simulink library "ammclib_bam"  (Simulink 9.3)
settings: Solver=VariableStepAuto  StartTime=0.0  StopTime=10.0  RelTol=1e-3
undefined symbols (not defined in the file): f16A1, f16A2, f16ADCMaxError, f16B0, f16B1, f16B2, f16C1, f16CC1, f16CC1sc, f16CC1sc_D, f16CC1sc_Q, f16CC2, f16CC2sc, f16CC2sc_D, f16CC2sc_Q, f16DerivGain, f16EGain, f16FiltCoef, f16HystOff, f16HystOn, f16IGain, f16IntegGain, f16IntegGainFW, f16IntegGainQ, f16Kd, f16Kq, f16Limit, f16LowerLimit, f16LowerLimit_D, f16LowerLimit_Q, f16LowerLimitFW, f16LowerLimitQ, f16ModIndex, f16OutValOff, f16OutValOn, f16PropGain, f16PropGainFW, f16PropGainQ, f16RampDown, f16RampUp, f16UGain, f16UpperLimit, f16UpperLimit_D, f16UpperLimit_Q, f16UpperLimitFW, f16UpperLimitQ, f16WIGain, f32A1, f32A2, f32ADCMaxError, f32B0, f32B1, f32B2, f32C1, f32CC1, f32CC1sc, f32CC1sc_D, f32CC1sc_Q, f32CC2, f32CC2sc ... (+62)
(part 2 of 15)

== system ammclib_bam/AMCLIB/F16 ==
  AMCLIB_BemfObsrvDQ_F16 : Subsystem  TreatAsAtomicUnit=on  mask(AMCLIB_BemfObsrvDQ_F16){showStates=Hide (faster execution), resetStatesEnable=Pre-set according to the first set of inputs after reset, f16IGain=0, f16UGain=0, f16WIGain=0, f16EGain=0, s16Shift=0, f16CC1sc_D=0, f16CC2sc_D=0, f16UpperLimit_D=0, f16LowerLimit_D=0, f16CC1sc_Q=0, f16CC2sc_Q=0, f16UpperLimit_Q=0, f16LowerLimit_Q=0, u16NShift=0}
      mask prompts: showStates "Show internal states"; resetStatesEnable "Internal state after reset"; f16IGain "f16IGain (Scaled RL circuit constant)"; f16UGain "f16UGain (Scaled voltage cross-coupling constant)"; f16WIGain "f16WIGain (Scaled angular velocity cross-coupling constant)"; f16EGain "f16EGain (Scaled back-EMF cross-coupling constant)"; s16Shift "s16Shift (Scaling bitwise shift applied to all cross-coupling constants)"; f16CC1sc_D "f16CC1sc_D (CC1 coefficient of the D-axis PI controller)"; f16CC2sc_D "f16CC2sc_D (CC2 coefficient of the D-axis PI controller)"; f16UpperLimit_D "f16UpperLimit_D (Upper Limit of the D-axis PI controller)"; f16LowerLimit_D "f16LowerLimit_D (Lower Limit of the D-axis PI controller)"; f16CC1sc_Q "f16CC1sc_Q (CC1 coefficient of the Q-axis PI controller)"; f16CC2sc_Q "f16CC2sc_Q (CC2 coefficient of the Q-axis PI controller)"; f16UpperLimit_Q "f16UpperLimit_Q (Upper Limit of the Q-axis PI controller)"; f16LowerLimit_Q "f16LowerLimit_Q (Lower Limit of the Q-axis PI controller)"; u16NShift "u16NShift (Scaling bitwise shift applied to the controller coefficients)"
      mask help: PMSM back-EMF observer DQ in 16-bit fixed-point fractional implementation. This block supports re-initialization of the internal state during simulation. If the block is reset, the observer will align with the motor's position and speed measured in the next time step. This allows seamless on-the-fly transition to the closed-loop control. Refer to the AMMCLIB User's Guide for further details.
      mask init:
      | if ~evalin('base','exist(''tS8'',''var'')')
      |   if (2 ~= exist('SWLIBS_Typedefs.mat','file'))
      |       error('File SWLIBS_Typedefs.mat is not on the Matlab path. Please add the AMMCLIB "bam" folder in the Matlab Search Path.');
      |   else
      |       evalin('base', 'load(''SWLIBS_Typedefs.mat'')');
      |   end
      | end
      | if showStates == 1
      |     % hidden state variables
      |     if strcmp(get_param([gcb '/f16IGain'], 'BlockType'), 'Inport')
      |         posblk = get_param(gcb, 'Position');
      | 
      |         pos = get_param(    [gcb, '/f16IGain'], 'Position');
      |         orient = get_param( [gcb, '/f16IGain'], 'Orientation');
      |         delete_block(       [gcb, '/f16IGain']);
      |         add_block('built-in/Ground', [gcb, '/f16IGain'], 'Position', pos, 'Orientation', orient);
      | 
      |         pos = get_param(    [gcb, '/f16UGain'], 'Position');
      |         orient = get_param( [gcb, '/f16UGain'], 'Orientation');
      |         delete_block(       [gcb, '/f16UGain']);
      |         add_block('built-in/Ground', [gcb, '/f16UGain'], 'Position', pos, 'Orientation', orient);
      | 
      |         pos = get_param(    [gcb, '/f16WIGain'], 'Position');
      |         orient = get_param( [gcb, '/f16WIGain'], 'Orientation');
      |         delete_block(       [gcb, '/f16WIGain']);
      |         add_block('built-in/Ground', [gcb, '/f16WIGain'], 'Position', pos, 'Orientation', orient);
      | 
      |         pos = get_param(    [gcb, '/f16EGain'], 'Position');
      |         orient = get_param( [gcb, '/f16EGain'], 'Orientation');
      |         delete_block(       [gcb, '/f16EGain']);
      |         add_block('built-in/Ground', [gcb, '/f16EGain'], 'Position', pos, 'Orientation', orient);
      | 
      |         pos = get_param(    [gcb, '/s16Shift'], 'Position');
      |         orient = get_param( [gcb, '/s16Shift'], 'Orientation');
      |         delete_block(       [gcb, '/s16Shift']);
      |         add_block('built-in/Ground', [gcb, '/s16Shift'], 'Position', pos, 'Orientation', orient);
      | 
      |         pos = get_param(    [gcb, '/f16CC1sc_D'], 'Position');
      |         orient = get_param( [gcb, '/f16CC1sc_D'], 'Orientation');
      |         delete_block(       [gcb, '/f16CC1sc_D']);
      |         add_block('built-in/Ground', [gcb, '/f16CC1sc_D'], 'Position', pos, 'Orientation', orient);
      | 
      |         pos = get_param(    [gcb, '/f16CC2sc_D'], 'Position');
      |         orient = get_param( [gcb, '/f16CC2sc_D'], 'Orientation');
      |         delete_block(       [gcb, '/f16CC2sc_D']);
      |         add_block('built-in/Ground', [gcb, '/f16CC2sc_D'], 'Position', pos, 'Orientation', orient);
      | 
      |         pos = get_param(    [gcb, '/f16UpperLimit_D'], 'Position');
      |         orient = get_param( [gcb, '/f16UpperLimit_D'], 'Orientation');
      |         delete_block(       [gcb, '/f16UpperLimit_D']);
      |         add_block('built-in/Ground', [gcb, '/f16UpperLimit_D'], 'Position', pos, 'Orientation', orient);
      | 
      |         pos = get_param(    [gcb, '/f16LowerLimit_D'], 'Position');
      |         orient = get_param( [gcb, '/f16LowerLimit_D'], 'Orientation');
      |         delete_block(       [gcb, '/f16LowerLimit_D']);
      |         add_block('built-in/Ground', [gcb, '/f16LowerLimit_D'], 'Position', pos, 'Orientation', orient);
      | 
      |         pos = get_param(    [gcb, '/f16CC1sc_Q'], 'Position');
      |         orient = get_param( [gcb, '/f16CC1sc_Q'], 'Orientation');
      |         delete_block(       [gcb, '/f16CC1sc_Q']);
      |         add_block('built-in/Ground', [gcb, '/f16CC1sc_Q'], 'Position', pos, 'Orientation', orient);
      | 
      |         pos = get_param(    [gcb, '/f16CC2sc_Q'], 'Position');
      |         orient = get_param( [gcb, '/f16CC2sc_Q'], 'Orientation');
      |         delete_block(       [gcb, '/f16CC2sc_Q']);
      |         add_block('built-in/Ground', [gcb, '/f16CC2sc_Q'], 'Position', pos, 'Orientation', orient);
      | 
      |         pos = get_param(    [gcb, '/f16UpperLimit_Q'], 'Position');
      |         orient = get_param( [gcb, '/f16UpperLimit_Q'], 'Orientation');
      |         delete_block(       [gcb, '/f16UpperLimit_Q']);
      |         add_block('built-in/Ground', [gcb, '/f16UpperLimit_Q'], 'Position', pos, 'Orientation', orient);
      | 
      |         pos = get_param(    [gcb, '/f16LowerLimit_Q'], 'Position');
      |         orient = get_param( [gcb, '/f16LowerLimit_Q'], 'Orientation');
      |         delete_block(       [gcb, '/f16LowerLimit_Q']);
      |         add_block('built-in/Ground', [gcb, '/f16LowerLimit_Q'], 'Position', pos, 'Orientation', orient);
      | 
      |         pos = get_param(    [gcb, '/u16NShift'], 'Position');
      |         orient = get_param( [gcb, '/u16NShift'], 'Orientation');
      |         delete_block(       [gcb, '/u16NShift']);
      |         add_block('built-in/Ground', [gcb, '/u16NShift'], 'Position', pos, 'Orientation', orient);
      | 
      |         pos = get_param(    [gcb, '/f32Acc_D'], 'Position');
      |         orient = get_param( [gcb, '/f32Acc_D'], 'Orientation');
      |         delete_block(       [gcb, '/f32Acc_D']);
      |         add_block('built-in/Ground', [gcb, '/f32Acc_D'], 'Position', pos, 'Orientation', orient);
      | 
      |         pos = get_param(    [gcb, '/f16InErrK1_D'], 'Position');
      |         orient = get_param( [gcb, '/f16InErrK1_D'], 'Orientation');
      |         delete_block(       [gcb, '/f16InErrK1_D']);
      |         add_block('built-in/Ground', [gcb, '/f16InErrK1_D'], 'Position', pos, 'Orientation', orient);
      | 
      |         pos = get_param(    [gcb, '/f32Acc_Q'], 'Position');
      |         orient = get_param( [gcb, '/f32Acc_Q'], 'Orientation');
      |         delete_block(       [gcb, '/f32Acc_Q']);
      |         add_block('built-in/Ground', [gcb, '/f32Acc_Q'], 'Position', pos, 'Orientation', orient);
      | 
      |         pos = get_param(    [gcb, '/f16InErrK1_Q'], 'Position');
      |         orient = get_param( [gcb, '/f16InErrK1_Q'], 'Orientation');
      |         delete_block(       [gcb, '/f16InErrK1_Q']);
      |         add_block('built-in/Ground', [gcb, '/f16InErrK1_Q'], 'Position', pos, 'Orientation', orient);
      | 
      |         pos = get_param(    [gcb, '/f32IObsrvIn_1L_D'], 'Position');
      |         orient = get_param( [gcb, '/f32IObsrvIn_1L_D'], 'Orientation');
      |         delete_block(       [gcb, '/f32IObsrvIn_1L_D']);
      |         add_block('built-in/Ground', [gcb, '/f32IObsrvIn_1L_D'], 'Position', pos, 'Orientation', orient);
      | 
      |         pos = get_param(    [gcb, '/f16IObsrvIn_1H_D'], 'Position');
      |         orient = get_param( [gcb, '/f16IObsrvIn_1H_D'], 'Orientation');
      |         delete_block(       [gcb, '/f16IObsrvIn_1H_D']);
      |         add_block('built-in/Ground', [gcb, '/f16IObsrvIn_1H_D'], 'Position', pos, 'Orientation', orient);
      | 
      |         pos = get_param(    [gcb, '/f32IObsrvIn_1L_Q'], 'Position');
      |         orient = get_param( [gcb, '/f32IObsrvIn_1L_Q'], 'Orientation');
      |         delete_block(       [gcb, '/f32IObsrvIn_1L_Q']);
      |         add_block('built-in/Ground', [gcb, '/f32IObsrvIn_1L_Q'], 'Position', pos, 'Orientation', orient);
      | 
      |         pos = get_param(    [gcb, '/f16IObsrvIn_1H_Q'], 'Position');
      |         orient = get_param( [gcb, '/f16IObsrvIn_1H_Q'], 'Orientation');
      |         delete_block(       [gcb, '/f16IObsrvIn_1H_Q']);
      |         add_block('built-in/Ground', [gcb, '/f16IObsrvIn_1H_Q'], 'Position', pos, 'Orientation', orient);
      | 
      |         pos = get_param(    [gcb, '/f32IObsrv_D'], 'Position');
      |         orient = get_param( [gcb, '/f32IObsrv_D'], 'Orientation');
      |         delete_block(       [gcb, '/f32IObsrv_D']);
      |         add_block('built-in/Ground', [gcb, '/f32IObsrv_D'], 'Position', pos, 'Orientation', orient);
      | 
      |         pos = get_param(    [gcb, '/f32IObsrv_Q'], 'Position');
      |         orient = get_param( [gcb, '/f32IObsrv_Q'], 'Orientation');
      |         delete_block(       [gcb, '/f32IObsrv_Q']);
      |         add_block('built-in/Ground', [gcb, '/f32IObsrv_Q'], 'Position', pos, 'Orientation', orient);
      | 
      | 
      |         pos = get_param(    [gcb '/f16EObsrv_D_Out'], 'Position');
      |         orient = get_param( [gcb '/f16EObsrv_D_Out'], 'Orientation');
      |         delete_block(       [gcb '/f16EObsrv_D_Out']);
      |         add_block('built-in/Terminator', [gcb '/f16EObsrv_D_Out'], 'Position', pos, 'Orientation', orient);
      | 
      |         pos = get_param(    [gcb '/f16EObsrv_Q_Out'], 'Position');
      |         orient = get_param( [gcb '/f16EObsrv_Q_Out'], 'Orientation');
      |         delete_block(       [gcb '/f16EObsrv_Q_Out']);
      |         add_block('built-in/Terminator', [gcb '/f16EObsrv_Q_Out'], 'Position', pos, 'Orientation', orient);
      | 
      |         pos = get_param(    [gcb '/f32Acc_D_Out'], 'Position');
      |         orient = get_param( [gcb '/f32Acc_D_Out'], 'Orientation');
      |         delete_block(       [gcb '/f32Acc_D_Out']);
      |         add_block('built-in/Terminator', [gcb '/f32Acc_D_Out'], 'Position', pos, 'Orientation', orient);
      | 
      |         pos = get_param(    [gcb '/f16InErrK1_D_Out'], 'Position');
      |         orient = get_param( [gcb '/f16InErrK1_D_Out'], 'Orientation');
      |         delete_block(       [gcb '/f16InErrK1_D_Out']);
      |         add_block('built-in/Terminator', [gcb '/f16InErrK1_D_Out'], 'Position', pos, 'Orientation', orient);
      | 
      |         pos = get_param(    [gcb '/f32Acc_Q_Out'], 'Position');
      |         orient = get_param( [gcb '/f32Acc_Q_Out'], 'Orientation');
      |         delete_block(       [gcb '/f32Acc_Q_Out']);
      |         add_block('built-in/Terminator', [gcb '/f32Acc_Q_Out'], 'Position', pos, 'Orientation', orient);
      | 
      |         pos = get_param(    [gcb '/f16InErrK1_Q_Out'], 'Position');
      |         orient = get_param( [gcb '/f16InErrK1_Q_Out'], 'Orientation');
      |         delete_block(       [gcb '/f16InErrK1_Q_Out']);
      |         add_block('built-in/Terminator', [gcb '/f16InErrK1_Q_Out'], 'Position', pos, 'Orientation', orient);
      | 
      |         pos = get_param(    [gcb '/f32IObsrvIn_1L_D_Out'], 'Position');
      |         orient = get_param( [gcb '/f32IObsrvIn_1L_D_Out'], 'Orientation');
      |         delete_block(       [gcb '/f32IObsrvIn_1L_D_Out']);
      |         add_block('built-in/Terminator', [gcb '/f32IObsrvIn_1L_D_Out'], 'Position', pos, 'Orientation', orient);
      | 
      |         pos = get_param(    [gcb '/f16IObsrvIn_1H_D_Out'], 'Position');
      |         orient = get_param( [gcb '/f16IObsrvIn_1H_D_Out'], 'Orientation');
      |         delete_block(       [gcb '/f16IObsrvIn_1H_D_Out']);
      |         add_block('built-in/Terminator', [gcb '/f16IObsrvIn_1H_D_Out'], 'Position', pos, 'Orientation', orient);
      | 
      |         pos = get_param(    [gcb '/f32IObsrvIn_1L_Q_Out'], 'Position');
      |         orient = get_param( [gcb '/f32IObsrvIn_1L_Q_Out'], 'Orientation');
      |         delete_block(       [gcb '/f32IObsrvIn_1L_Q_Out']);
      |         add_block('built-in/Terminator', [gcb '/f32IObsrvIn_1L_Q_Out'], 'Position', pos, 'Orientation', orient);
      | 
      |         pos = get_param(    [gcb '/f16IObsrvIn_1H_Q_Out'], 'Position');
      |         orient = get_param( [gcb '/f16IObsrvIn_1H_Q_Out'], 'Orientation');
      |         delete_block(       [gcb '/f16IObsrvIn_1H_Q_Out']);
      |         add_block('built-in/Terminator', [gcb '/f16IObsrvIn_1H_Q_Out'], 'Position', pos, 'Orientation', orient);
      | 
      |         pos = get_param(    [gcb '/f32IObsrv_D_Out'], 'Position');
      |         orient = get_param( [gcb '/f32IObsrv_D_Out'], 'Orientation');
      |         delete_block(       [gcb '/f32IObsrv_D_Out']);
      |         add_block('built-in/Terminator', [gcb '/f32IObsrv_D_Out'], 'Position', pos, 'Orientation', orient);
      | 
      |         pos = get_param(    [gcb '/f32IObsrv_Q_Out'], 'Position');
      |         orient = get_param( [gcb '/f32IObsrv_Q_Out'], 'Orientation');
      |         delete_block(       [gcb '/f32IObsrv_Q_Out']);
      |         add_block('built-in/Terminator', [gcb '/f32IObsrv_Q_Out'], 'Position', pos, 'Orientation', orient);
      | 
      | 
      |         set_param([gcb '/pIAB'], 'Port', '1');
      |         set_param([gcb '/pUAB'], 'Port', '2');
      |         set_param([gcb '/f16Velocity'], 'Port', '3');
      |         set_param([gcb '/f16Phase'], 'Port', '4');
      | 
      |         set_param([gcb '/f16PhaseErr'], 'Port', '1');
      | 
      |         set_param(gcb,'MaskEnables',{'on','on','on','on','on','on','on','on','on','on','on','on','on','on','on','on'});
      | 
      |         if (posblk(4) - posblk(2)) > 125
      |           height = 125;
      |           set_param(gcb,'Position',[posblk(1), posblk(2), posblk(3), posblk(2)+height])
      |         end
      |     end
      | else
      |     % shown state variables
      |     if strcmp(get_param([gcb '/f16IGain'], 'BlockType'), 'Ground')
      |         posblk = get_param(gcb, 'Position');
      | 
      |         pos = get_param(    [gcb, '/f16IGain'], 'Position');
      |         orient = get_param( [gcb, '/f16IGain'], 'Orientation');
      |         delete_block(       [gcb, '/f16IGain']);
      |         add_block('built-in/Inport', [gcb, '/f16IGain'], 'Position', pos, 'Orientation', orient, 'OutDataTypeStr', 'int16');
      | 
      |         pos = get_param(    [gcb, '/f16UGain'], 'Position');
      |         orient = get_param( [gcb, '/f16UGain'], 'Orientation');
      |         delete_block(       [gcb, '/f16UGain']);
      |         add_block('built-in/Inport', [gcb, '/f16UGain'], 'Position', pos, 'Orientation', orient, 'OutDataTypeStr', 'int16');
      | 
      |         pos = get_param(    [gcb, '/f16WIGain'], 'Position');
      |         orient = get_param( [gcb, '/f16WIGain'], 'Orientation');
      |         delete_block(       [gcb, '/f16WIGain']);
      |         add_block('built-in/Inport', [gcb, '/f16WIGain'], 'Position', pos, 'Orientation', orient, 'OutDataTypeStr', 'int16');
      | 
      |         pos = get_param(    [gcb, '/f16EGain'], 'Position');
      |         orient = get_param( [gcb, '/f16EGain'], 'Orientation');
      |         delete_block(       [gcb, '/f16EGain']);
      |         add_block('built-in/Inport', [gcb, '/f16EGain'], 'Position', pos, 'Orientation', orient, 'OutDataTypeStr', 'int16');
      | 
      |         pos = get_param(    [gcb, '/s16Shift'], 'Position');
      |         orient = get_param( [gcb, '/s16Shift'], 'Orientation');
      |         delete_block(       [gcb, '/s16Shift']);
      |         add_block('built-in/Inport', [gcb, '/s16Shift'], 'Position', pos, 'Orientation', orient, 'OutDataTypeStr', 'int16');
      | 
      |         pos = get_param(    [gcb, '/f16CC1sc_D'], 'Position');
      |         orient = get_param( [gcb, '/f16CC1sc_D'], 'Orientation');
      |         delete_block(       [gcb, '/f16CC1sc_D']);
      |         add_block('built-in/Inport', [gcb, '/f16CC1sc_D'], 'Position', pos, 'Orientation', orient, 'OutDataTypeStr', 'int16');
      | 
      |         pos = get_param(    [gcb, '/f16CC2sc_D'], 'Position');
      |         orient = get_param( [gcb, '/f16CC2sc_D'], 'Orientation');
      |         delete_block(       [gcb, '/f16CC2sc_D']);
      |         add_block('built-in/Inport', [gcb, '/f16CC2sc_D'], 'Position', pos, 'Orientation', orient, 'OutDataTypeStr', 'int16');
      | 
      |         pos = get_param(    [gcb, '/f16UpperLimit_D'], 'Position');
      |         orient = get_param( [gcb, '/f16UpperLimit_D'], 'Orientation');
      |         delete_block(       [gcb, '/f16UpperLimit_D']);
      |         add_block('built-in/Inport', [gcb, '/f16UpperLimit_D'], 'Position', pos, 'Orientation', orient, 'OutDataTypeStr', 'int16');
      | 
      |         pos = get_param(    [gcb, '/f16LowerLimit_D'], 'Position');
      |         orient = get_param( [gcb, '/f16LowerLimit_D'], 'Orientation');
      |         delete_block(       [gcb, '/f16LowerLimit_D']);
      |         add_block('built-in/Inport', [gcb, '/f16LowerLimit_D'], 'Position', pos, 'Orientation', orient, 'OutDataTypeStr', 'int16');
      | 
      |         pos = get_param(    [gcb, '/f16CC1sc_Q'], 'Position');
      |         orient = get_param( [gcb, '/f16CC1sc_Q'], 'Orientation');
      |         delete_block(       [gcb, '/f16CC1sc_Q']);
      |         add_block('built-in/Inport', [gcb, '/f16CC1sc_Q'], 'Position', pos, 'Orientation', orient, 'OutDataTypeStr', 'int16');
      | 
      |         pos = get_param(    [gcb, '/f16CC2sc_Q'], 'Position');
      |         orient = get_param( [gcb, '/f16CC2sc_Q'], 'Orientation');
      |         delete_block(       [gcb, '/f16CC2sc_Q']);
      |         add_block('built-in/Inport', [gcb, '/f16CC2sc_Q'], 'Position', pos, 'Orientation', orient, 'OutDataTypeStr', 'int16');
      | 
      |         pos = get_param(    [gcb, '/f16UpperLimit_Q'], 'Position');
      |         orient = get_param( [gcb, '/f16UpperLimit_Q'], 'Orientation');
      |         delete_block(       [gcb, '/f16UpperLimit_Q']);
      |         add_block('built-in/Inport', [gcb, '/f16UpperLimit_Q'], 'Position', pos, 'Orientation', orient, 'OutDataTypeStr', 'int16');
      | 
      |         pos = get_param(    [gcb, '/f16LowerLimit_Q'], 'Position');
      |         orient = get_param( [gcb, '/f16LowerLimit_Q'], 'Orientation');
      |         delete_block(       [gcb, '/f16LowerLimit_Q']);
      |         add_block('built-in/Inport', [gcb, '/f16LowerLimit_Q'], 'Position', pos, 'Orientation', orient, 'OutDataTypeStr', 'int16');
      | 
      |         pos = get_param(    [gcb, '/u16NShift'], 'Position');
      |         orient = get_param( [gcb, '/u16NShift'], 'Orientation');
      |         delete_block(       [gcb, '/u16NShift']);
      |         add_block('built-in/Inport', [gcb, '/u16NShift'], 'Position', pos, 'Orientation', orient, 'OutDataTypeStr', 'uint16');
      | 
      |         pos = get_param(    [gcb, '/f32Acc_D'], 'Position');
      |         orient = get_param( [gcb, '/f32Acc_D'], 'Orientation');
      |         delete_block(       [gcb, '/f32Acc_D']);
      |         add_block('built-in/Inport', [gcb, '/f32Acc_D'], 'Position', pos, 'Orientation', orient, 'OutDataTypeStr', 'int32');
      | 
      |         pos = get_param(    [gcb, '/f16InErrK1_D'], 'Position');
      |         orient = get_param( [gcb, '/f16InErrK1_D'], 'Orientation');
      |         delete_block(       [gcb, '/f16InErrK1_D']);
      |         add_block('built-in/Inport', [gcb, '/f16InErrK1_D'], 'Position', pos, 'Orientation', orient, 'OutDataTypeStr', 'int16');
      | 
      |         pos = get_param(    [gcb, '/f32Acc_Q'], 'Position');
      |         orient = get_param( [gcb, '/f32Acc_Q'], 'Orientation');
      |         delete_block(       [gcb, '/f32Acc_Q']);
      |         add_block('built-in/Inport', [gcb, '/f32Acc_Q'], 'Position', pos, 'Orientation', orient, 'OutDataTypeStr', 'int32');
      | 
      |         pos = get_param(    [gcb, '/f16InErrK1_Q'], 'Position');
      |         orient = get_param( [gcb, '/f16InErrK1_Q'], 'Orientation');
      |         delete_block(       [gcb, '/f16InErrK1_Q']);
      |         add_block('built-in/Inport', [gcb, '/f16InErrK1_Q'], 'Position', pos, 'Orientation', orient, 'OutDataTypeStr', 'int16');
      | 
      |         pos = get_param(    [gcb, '/f32IObsrvIn_1L_D'], 'Position');
      |         orient = get_param( [gcb, '/f32IObsrvIn_1L_D'], 'Orientation');
      |         delete_block(       [gcb, '/f32IObsrvIn_1L_D']);
      |         add_block('built-in/Inport', [gcb, '/f32IObsrvIn_1L_D'], 'Position', pos, 'Orientation', orient, 'OutDataTypeStr', 'int32');
      | 
      |         pos = get_param(    [gcb, '/f16IObsrvIn_1H_D'], 'Position');
      |         orient = get_param( [gcb, '/f16IObsrvIn_1H_D'], 'Orientation');
      |         delete_block(       [gcb, '/f16IObsrvIn_1H_D']);
      |         add_block('built-in/Inport', [gcb, '/f16IObsrvIn_1H_D'], 'Position', pos, 'Orientation', orient, 'OutDataTypeStr', 'int16');
      | 
      |         pos = get_param(    [gcb, '/f32IObsrvIn_1L_Q'], 'Position');
      |         orient = get_param( [gcb, '/f32IObsrvIn_1L_Q'], 'Orientation');
      |         delete_block(       [gcb, '/f32IObsrvIn_1L_Q']);
      |         add_block('built-in/Inport', [gcb, '/f32IObsrvIn_1L_Q'], 'Position', pos, 'Orientation', orient, 'OutDataTypeStr', 'int32');
      | 
      |         pos = get_param(    [gcb, '/f16IObsrvIn_1H_Q'], 'Position');
      |         orient = get_param( [gcb, '/f16IObsrvIn_1H_Q'], 'Orientation');
      |         delete_block(       [gcb, '/f16IObsrvIn_1H_Q']);
      |         add_block('built-in/Inport', [gcb, '/f16IObsrvIn_1H_Q'], 'Position', pos, 'Orientation', orient, 'OutDataTypeStr', 'int16');
      | 
      |         pos = get_param(    [gcb, '/f32IObsrv_D'], 'Position');
      |         orient = get_param( [gcb, '/f32IObsrv_D'], 'Orientation');
      |         delete_block(       [gcb, '/f32IObsrv_D']);
      |         add_block('built-in/Inport', [gcb, '/f32IObsrv_D'], 'Position', pos, 'Orientation', orient, 'OutDataTypeStr', 'int32');
      | 
      |         pos = get_param(    [gcb, '/f32IObsrv_Q'], 'Position');
      |         orient = get_param( [gcb, '/f32IObsrv_Q'], 'Orientation');
      |         delete_block(       [gcb, '/f32IObsrv_Q']);
      |         add_block('built-in/Inport', [gcb, '/f32IObsrv_Q'], 'Position', pos, 'Orientation', orient, 'OutDataTypeStr', 'int32');
      | 
      | 
      |         pos = get_param(    [gcb '/f16EObsrv_D_Out'], 'Position');
      |         orient = get_param( [gcb '/f16EObsrv_D_Out'], 'Orientation');
      |         delete_block(       [gcb '/f16EObsrv_D_Out']);
      |         add_block('built-in/Outport', [gcb '/f16EObsrv_D_Out'], 'Position', pos, 'Orientation', orient);
      | 
      |         pos = get_param(    [gcb '/f16EObsrv_Q_Out'], 'Position');
      |         orient = get_param( [gcb '/f16EObsrv_Q_Out'], 'Orientation');
      |         delete_block(       [gcb '/f16EObsrv_Q_Out']);
      |         add_block('built-in/Outport', [gcb '/f16EObsrv_Q_Out'], 'Position', pos, 'Orientation', orient);
      | 
      |         pos = get_param(    [gcb '/f32Acc_D_Out'], 'Position');
      |         orient = get_param( [gcb '/f32Acc_D_Out'], 'Orientation');
      |         delete_block(       [gcb '/f32Acc_D_Out']);
      |         add_block('built-in/Outport', [gcb '/f32Acc_D_Out'], 'Position', pos, 'Orientation', orient);
      | 
      |         pos = get_param(    [gcb '/f16InErrK1_D_Out'], 'Position');
      |         orient = get_param( [gcb '/f16InErrK1_D_Out'], 'Orientation');
      |         delete_block(       [gcb '/f16InErrK1_D_Out']);
      |         add_block('built-in/Outport', [gcb '/f16InErrK1_D_Out'], 'Position', pos, 'Orientation', orient);
      | 
      |         pos = get_param(    [gcb '/f32Acc_Q_Out'], 'Position');
      |         orient = get_param( [gcb '/f32Acc_Q_Out'], 'Orientation');
      |         delete_block(       [gcb '/f32Acc_Q_Out']);
      |         add_block('built-in/Outport', [gcb '/f32Acc_Q_Out'], 'Position', pos, 'Orientation', orient);
      | 
      |         pos = get_param(    [gcb '/f16InErrK1_Q_Out'], 'Position');
      |         orient = get_param( [gcb '/f16InErrK1_Q_Out'], 'Orientation');
      |         delete_block(       [gcb '/f16InErrK1_Q_Out']);
      |         add_block('built-in/Outport', [gcb '/f16InErrK1_Q_Out'], 'Position', pos, 'Orientation', orient);
      | 
      |         pos = get_param(    [gcb '/f32IObsrvIn_1L_D_Out'], 'Position');
      |         orient = get_param( [gcb '/f32IObsrvIn_1L_D_Out'], 'Orientation');
      |         delete_block(       [gcb '/f32IObsrvIn_1L_D_Out']);
      |         add_block('built-in/Outport', [gcb '/f32IObsrvIn_1L_D_Out'], 'Position', pos, 'Orientation', orient);
      | 
      |         pos = get_param(    [gcb '/f16IObsrvIn_1H_D_Out'], 'Position');
      |         orient = get_param( [gcb '/f16IObsrvIn_1H_D_Out'], 'Orientation');
      |         delete_block(       [gcb '/f16IObsrvIn_1H_D_Out']);
      |         add_block('built-in/Outport', [gcb '/f16IObsrvIn_1H_D_Out'], 'Position', pos, 'Orientation', orient);
      | 
      |         pos = get_param(    [gcb '/f32IObsrvIn_1L_Q_Out'], 'Position');
      |         orient = get_param( [gcb '/f32IObsrvIn_1L_Q_Out'], 'Orientation');
      |         delete_block(       [gcb '/f32IObsrvIn_1L_Q_Out']);
      |         add_block('built-in/Outport', [gcb '/f32IObsrvIn_1L_Q_Out'], 'Position', pos, 'Orientation', orient);
      | 
      |         pos = get_param(    [gcb '/f16IObsrvIn_1H_Q_Out'], 'Position');
      |         orient = get_param( [gcb '/f16IObsrvIn_1H_Q_Out'], 'Orientation');
      |         delete_block(       [gcb '/f16IObsrvIn_1H_Q_Out']);
      |         add_block('built-in/Outport', [gcb '/f16IObsrvIn_1H_Q_Out'], 'Position', pos, 'Orientation', orient);
      | 
      |         pos = get_param(    [gcb '/f32IObsrv_D_Out'], 'Position');
      |         orient = get_param( [gcb '/f32IObsrv_D_Out'], 'Orientation');
      |         delete_block(       [gcb '/f32IObsrv_D_Out']);
      |         add_block('built-in/Outport', [gcb '/f32IObsrv_D_Out'], 'Position', pos, 'Orientation', orient);
      | 
      |         pos = get_param(    [gcb '/f32IObsrv_Q_Out'], 'Position');
      |         orient = get_param( [gcb '/f32IObsrv_Q_Out'], 'Orientation');
      |         delete_block(       [gcb '/f32IObsrv_Q_Out']);
      |         add_block('built-in/Outport', [gcb '/f32IObsrv_Q_Out'], 'Position', pos, 'Orientation', orient);
      | 
      | 
      |         set_param([gcb '/pIAB'], 'Port', '1');
      |         set_param([gcb '/pUAB'], 'Port', '2');
      |         set_param([gcb '/f16Velocity'], 'Port', '3');
      |         set_param([gcb '/f16Phase'], 'Port', '4');
      |         set_param([gcb '/f16IGain'], 'Port', '5');
      |         set_param([gcb '/f16UGain'], 'Port', '6');
      |         set_param([gcb '/f16WIGain'], 'Port', '7');
      |         set_param([gcb '/f16EGain'], 'Port', '8');
      |         set_param([gcb '/s16Shift'], 'Port', '9');
      |         set_param([gcb '/f16CC1sc_D'], 'Port', '10');
      |         set_param([gcb '/f16CC2sc_D'], 'Port', '11');
      |         set_param([gcb '/f16UpperLimit_D'], 'Port', '12');
      |         set_param([gcb '/f16LowerLimit_D'], 'Port', '13');
      |         set_param([gcb '/f16CC1sc_Q'], 'Port', '14');
      |         set_param([gcb '/f16CC2sc_Q'], 'Port', '15');
      |         set_param([gcb '/f16UpperLimit_Q'], 'Port', '16');
      |         set_param([gcb '/f16LowerLimit_Q'], 'Port', '17');
      |         set_param([gcb '/u16NShift'], 'Port', '18');
      |         set_param([gcb '/f32Acc_D'], 'Port', '19');
      |         set_param([gcb '/f16InErrK1_D'], 'Port', '20');
      |         set_param([gcb '/f32Acc_Q'], 'Port', '21');
      |         set_param([gcb '/f16InErrK1_Q'], 'Port', '22');
      |         set_param([gcb '/f32IObsrvIn_1L_D'], 'Port', '23');
      |         set_param([gcb '/f16IObsrvIn_1H_D'], 'Port', '24');
      |         set_param([gcb '/f32IObsrvIn_1L_Q'], 'Port', '25');
      |         set_param([gcb '/f16IObsrvIn_1H_Q'], 'Port', '26');
      |         set_param([gcb '/f32IObsrv_D'], 'Port', '27');
      |         set_param([gcb '/f32IObsrv_Q'], 'Port', '28');
      | 
      |         set_param([gcb '/f16PhaseErr'], 'Port', '1');
      |         set_param([gcb '/f16EObsrv_D_Out'], 'Port', '2');
      |         set_param([gcb '/f16EObsrv_Q_Out'], 'Port', '3');
      |         set_param([gcb '/f32Acc_D_Out'], 'Port', '4');
      |         set_param([gcb '/f16InErrK1_D_Out'], 'Port', '5');
      |         set_param([gcb '/f32Acc_Q_Out'], 'Port', '6');
      |         set_param([gcb '/f16InErrK1_Q_Out'], 'Port', '7');
      |         set_param([gcb '/f32IObsrvIn_1L_D_Out'], 'Port', '8');
      |         set_param([gcb '/f16IObsrvIn_1H_D_Out'], 'Port', '9');
      |         set_param([gcb '/f32IObsrvIn_1L_Q_Out'], 'Port', '10');
      |         set_param([gcb '/f16IObsrvIn_1H_Q_Out'], 'Port', '11');
      |         set_param([gcb '/f32IObsrv_D_Out'], 'Port', '12');
      |         set_param([gcb '/f32IObsrv_Q_Out'], 'Port', '13');
      | 
      |         set_param(gcb,'MaskEnables',{'on','on','off','off','off','off','off','off','off','off','off','off','off','off','off','off'});
      | 
      |         if (posblk(4) - posblk(2)) < 725
      |           height = 725;
      |           set_param(gcb,'Position',[posblk(1), posblk(2), posblk(3), posblk(2)+height])
      |         end
      |     end
      | end
      settings: RTWSystemCode=Inline
      mask TypeOptions showStates: Hide (faster execution) | Show (allows debugging; connect feedback loops manually)
      mask Callback showStates:
      | maskStr = get_param(gcb,'showStates');
      | if strcmp(maskStr,'Hide (faster execution)'),
      |     set_param(gcb,'MaskEnables',{'on','on','on','on','on','on','on','on','on','on','on','on','on','on','on','on'});
      | else
      |     set_param(gcb,'MaskEnables',{'on','on','off','off','off','off','off','off','off','off','off','off','off','off','off','off'});
      | end
      mask TypeOptions resetStatesEnable: Pre-set according to the first set of inputs after reset | Clear to zero
      mask Display:
      | color('black');
      | pos = get_param(gcb, 'Position');
      | width = pos(3) - pos(1);
      | height = pos(4) - pos(2);
      | tX=width/2;
      | tY=height - 25;
      | color('black');
      | text(tX,tY, 'AMCLIB_BemfObsrvDQ_F16', 'horizontalAlignment', 'center');
      | if showStates == 2
      |   color('red');
      |   text(tX,tY - 20, ['debugging mode' char(13) char(10) '(limited performance)'], 'horizontalAlignment', 'center');
      | end
  AMCLIB_CurrentLoop_F16 : Subsystem  TreatAsAtomicUnit=on  mask(AMCLIB_CurrentLoop_F16){showStates=Hide (faster execution), resetStatesEnable=Pre-set according to the first set of inputs after reset, f16CC1sc_D=0, f16CC2sc_D=0, u16NShift_D=0, f16CC1sc_Q=0, f16CC2sc_Q=0, u16NShift_Q=0}
      mask prompts: showStates "Show internal states"; resetStatesEnable "Internal state after reset"; f16CC1sc_D "f16CC1sc_D (CC1 coefficient of the D-axis PI controller)"; f16CC2sc_D "f16CC2sc_D (CC2 coefficient of the D-axis PI controller)"; u16NShift_D "u16NShift_D (Scaling bitwise shift applied to the D-axis controller coefficients)"; f16CC1sc_Q "f16CC1sc_Q (CC1 coefficient of the Q-axis PI controller)"; f16CC2sc_Q "f16CC2sc_Q (CC2 coefficient of the Q-axis PI controller)"; u16NShift_Q "u16NShift_Q (Scaling bitwise shift applied to the Q-axis controller coefficients)"
      mask help: Current control loop of the PMSM field-oriented control algorithm in 16-bit fixed-point fractional implementation. This block supports re-initialization of the internal state during simulation. If the block is reset, the outputs of the PI controllers will be aligned with the inputs f16ControllerPIrAWDOut_preset and f16ControllerPIrAWQOut_preset. Refer to the AMMCLIB User's Guide for further details.
      mask init:
      | if ~evalin('base','exist(''tS8'',''var'')')
      |   if (2 ~= exist('SWLIBS_Typedefs.mat','file'))
      |       error('File SWLIBS_Typedefs.mat is not on the Matlab path. Please add the AMMCLIB "bam" folder in the Matlab Search Path.');
      |   else
      |       evalin('base', 'load(''SWLIBS_Typedefs.mat'')');
      |   end
      | end
      | if showStates == 1
      |     % hidden state variables
      |     if strcmp(get_param([gcb '/f16CC1sc_D'], 'BlockType'), 'Inport')
      |         posblk = get_param(gcb, 'Position');
      | 
      |         pos = get_param(    [gcb, '/f16CC1sc_D'], 'Position');
      |         orient = get_param( [gcb, '/f16CC1sc_D'], 'Orientation');
      |         delete_block(       [gcb, '/f16CC1sc_D']);
      |         add_block('built-in/Ground', [gcb, '/f16CC1sc_D'], 'Position', pos, 'Orientation', orient);
      | 
      |         pos = get_param(    [gcb, '/f16CC2sc_D'], 'Position');
      |         orient = get_param( [gcb, '/f16CC2sc_D'], 'Orientation');
      |         delete_block(       [gcb, '/f16CC2sc_D']);
      |         add_block('built-in/Ground', [gcb, '/f16CC2sc_D'], 'Position', pos, 'Orientation', orient);
      | 
      |         pos = get_param(    [gcb, '/u16NShift_D'], 'Position');
      |         orient = get_param( [gcb, '/u16NShift_D'], 'Orientation');
      |         delete_block(       [gcb, '/u16NShift_D']);
      |         add_block('built-in/Ground', [gcb, '/u16NShift_D'], 'Position', pos, 'Orientation', orient);
      | 
      |         pos = get_param(    [gcb, '/f16CC1sc_Q'], 'Position');
      |         orient = get_param( [gcb, '/f16CC1sc_Q'], 'Orientation');
      |         delete_block(       [gcb, '/f16CC1sc_Q']);
      |         add_block('built-in/Ground', [gcb, '/f16CC1sc_Q'], 'Position', pos, 'Orientation', orient);
      | 
      |         pos = get_param(    [gcb, '/f16CC2sc_Q'], 'Position');
      |         orient = get_param( [gcb, '/f16CC2sc_Q'], 'Orientation');
      |         delete_block(       [gcb, '/f16CC2sc_Q']);
      |         add_block('built-in/Ground', [gcb, '/f16CC2sc_Q'], 'Position', pos, 'Orientation', orient);
      | 
      |         pos = get_param(    [gcb, '/u16NShift_Q'], 'Position');
      |         orient = get_param( [gcb, '/u16NShift_Q'], 'Orientation');
      |         delete_block(       [gcb, '/u16NShift_Q']);
      |         add_block('built-in/Ground', [gcb, '/u16NShift_Q'], 'Position', pos, 'Orientation', orient);
      | 
      |         pos = get_param(    [gcb, '/f32Acc_D'], 'Position');
      |         orient = get_param( [gcb, '/f32Acc_D'], 'Orientation');
      |         delete_block(       [gcb, '/f32Acc_D']);
      |         add_block('built-in/Ground', [gcb, '/f32Acc_D'], 'Position', pos, 'Orientation', orient);
      | 
      |         pos = get_param(    [gcb, '/f16InErrK1_D'], 'Position');
      |         orient = get_param( [gcb, '/f16InErrK1_D'], 'Orientation');
      |         delete_block(       [gcb, '/f16InErrK1_D']);
      |         add_block('built-in/Ground', [gcb, '/f16InErrK1_D'], 'Position', pos, 'Orientation', orient);
      | 
      |         pos = get_param(    [gcb, '/f32Acc_Q'], 'Position');
      |         orient = get_param( [gcb, '/f32Acc_Q'], 'Orientation');
      |         delete_block(       [gcb, '/f32Acc_Q']);
      |         add_block('built-in/Ground', [gcb, '/f32Acc_Q'], 'Position', pos, 'Orientation', orient);
      | 
      |         pos = get_param(    [gcb, '/f16InErrK1_Q'], 'Position');
      |         orient = get_param( [gcb, '/f16InErrK1_Q'], 'Orientation');
      |         delete_block(       [gcb, '/f16InErrK1_Q']);
      |         add_block('built-in/Ground', [gcb, '/f16InErrK1_Q'], 'Position', pos, 'Orientation', orient);
      | 
      | 
      |         pos = get_param(    [gcb '/f32Acc_D_Out'], 'Position');
      |         orient = get_param( [gcb '/f32Acc_D_Out'], 'Orientation');
      |         delete_block(       [gcb '/f32Acc_D_Out']);
      |         add_block('built-in/Terminator', [gcb '/f32Acc_D_Out'], 'Position', pos, 'Orientation', orient);
      | 
      |         pos = get_param(    [gcb '/f16InErrK1_D_Out'], 'Position');
      |         orient = get_param( [gcb '/f16InErrK1_D_Out'], 'Orientation');
      |         delete_block(       [gcb '/f16InErrK1_D_Out']);
      |         add_block('built-in/Terminator', [gcb '/f16InErrK1_D_Out'], 'Position', pos, 'Orientation', orient);
      | 
      |         pos = get_param(    [gcb '/f32Acc_Q_Out'], 'Position');
      |         orient = get_param( [gcb '/f32Acc_Q_Out'], 'Orientation');
      |         delete_block(       [gcb '/f32Acc_Q_Out']);
      |         add_block('built-in/Terminator', [gcb '/f32Acc_Q_Out'], 'Position', pos, 'Orientation', orient);
      | 
      |         pos = get_param(    [gcb '/f16InErrK1_Q_Out'], 'Position');
      |         orient = get_param( [gcb '/f16InErrK1_Q_Out'], 'Orientation');
      |         delete_block(       [gcb '/f16InErrK1_Q_Out']);
      |         add_block('built-in/Terminator', [gcb '/f16InErrK1_Q_Out'], 'Position', pos, 'Orientation', orient);
      | 
      | 
      |         set_param([gcb '/f16UDcBus'], 'Port', '1');
      |         set_param([gcb '/pIDQReq'], 'Port', '2');
      |         set_param([gcb '/pIDQFbck'], 'Port', '3');
      |         set_param([gcb '/f16ControllerPIrAWDOut_preset'], 'Port', '4');
      |         set_param([gcb '/f16ControllerPIrAWQOut_preset'], 'Port', '5');
      | 
      |         set_param([gcb '/pUDQReq'], 'Port', '1');
      | 
      |         set_param(gcb,'MaskEnables',{'on','on','on','on','on','on','on','on'});
      | 
      |         if (posblk(4) - posblk(2)) > 150
      |           height = 150;
      |           set_param(gcb,'Position',[posblk(1), posblk(2), posblk(3), posblk(2)+height])
      |         end
      |     end
      | else
      |     % shown state variables
      |     if strcmp(get_param([gcb '/f16CC1sc_D'], 'BlockType'), 'Ground')
      |         posblk = get_param(gcb, 'Position');
      | 
      |         pos = get_param(    [gcb, '/f16CC1sc_D'], 'Position');
      |         orient = get_param( [gcb, '/f16CC1sc_D'], 'Orientation');
      |         delete_block(       [gcb, '/f16CC1sc_D']);
      |         add_block('built-in/Inport', [gcb, '/f16CC1sc_D'], 'Position', pos, 'Orientation', orient, 'OutDataTypeStr', 'int16');
      | 
      |         pos = get_param(    [gcb, '/f16CC2sc_D'], 'Position');
      |         orient = get_param( [gcb, '/f16CC2sc_D'], 'Orientation');
      |         delete_block(       [gcb, '/f16CC2sc_D']);
      |         add_block('built-in/Inport', [gcb, '/f16CC2sc_D'], 'Position', pos, 'Orientation', orient, 'OutDataTypeStr', 'int16');
      | 
      |         pos = get_param(    [gcb, '/u16NShift_D'], 'Position');
      |         orient = get_param( [gcb, '/u16NShift_D'], 'Orientation');
      |         delete_block(       [gcb, '/u16NShift_D']);
      |         add_block('built-in/Inport', [gcb, '/u16NShift_D'], 'Position', pos, 'Orientation', orient, 'OutDataTypeStr', 'uint16');
      | 
      |         pos = get_param(    [gcb, '/f16CC1sc_Q'], 'Position');
      |         orient = get_param( [gcb, '/f16CC1sc_Q'], 'Orientation');
      |         delete_block(       [gcb, '/f16CC1sc_Q']);
      |         add_block('built-in/Inport', [gcb, '/f16CC1sc_Q'], 'Position', pos, 'Orientation', orient, 'OutDataTypeStr', 'int16');
      | 
      |         pos = get_param(    [gcb, '/f16CC2sc_Q'], 'Position');
      |         orient = get_param( [gcb, '/f16CC2sc_Q'], 'Orientation');
      |         delete_block(       [gcb, '/f16CC2sc_Q']);
      |         add_block('built-in/Inport', [gcb, '/f16CC2sc_Q'], 'Position', pos, 'Orientation', orient, 'OutDataTypeStr', 'int16');
      | 
      |         pos = get_param(    [gcb, '/u16NShift_Q'], 'Position');
      |         orient = get_param( [gcb, '/u16NShift_Q'], 'Orientation');
      |         delete_block(       [gcb, '/u16NShift_Q']);
      |         add_block('built-in/Inport', [gcb, '/u16NShift_Q'], 'Position', pos, 'Orientation', orient, 'OutDataTypeStr', 'uint16');
      | 
      |         pos = get_param(    [gcb, '/f32Acc_D'], 'Position');
      |         orient = get_param( [gcb, '/f32Acc_D'], 'Orientation');
      |         delete_block(       [gcb, '/f32Acc_D']);
      |         add_block('built-in/Inport', [gcb, '/f32Acc_D'], 'Position', pos, 'Orientation', orient, 'OutDataTypeStr', 'int32');
      | 
      |         pos = get_param(    [gcb, '/f16InErrK1_D'], 'Position');
      |         orient = get_param( [gcb, '/f16InErrK1_D'], 'Orientation');
      |         delete_block(       [gcb, '/f16InErrK1_D']);
      |         add_block('built-in/Inport', [gcb, '/f16InErrK1_D'], 'Position', pos, 'Orientation', orient, 'OutDataTypeStr', 'int16');
      | 
      |         pos = get_param(    [gcb, '/f32Acc_Q'], 'Position');
      |         orient = get_param( [gcb, '/f32Acc_Q'], 'Orientation');
      |         delete_block(       [gcb, '/f32Acc_Q']);
      |         add_block('built-in/Inport', [gcb, '/f32Acc_Q'], 'Position', pos, 'Orientation', orient, 'OutDataTypeStr', 'int32');
      | 
      |         pos = get_param(    [gcb, '/f16InErrK1_Q'], 'Position');
      |         orient = get_param( [gcb, '/f16InErrK1_Q'], 'Orientation');
      |         delete_block(       [gcb, '/f16InErrK1_Q']);
      |         add_block('built-in/Inport', [gcb, '/f16InErrK1_Q'], 'Position', pos, 'Orientation', orient, 'OutDataTypeStr', 'int16');
      | 
      | 
      |         pos = get_param(    [gcb '/f32Acc_D_Out'], 'Position');
      |         orient = get_param( [gcb '/f32Acc_D_Out'], 'Orientation');
      |         delete_block(       [gcb '/f32Acc_D_Out']);
      |         add_block('built-in/Outport', [gcb '/f32Acc_D_Out'], 'Position', pos, 'Orientation', orient);
      | 
      |         pos = get_param(    [gcb '/f16InErrK1_D_Out'], 'Position');
      |         orient = get_param( [gcb '/f16InErrK1_D_Out'], 'Orientation');
      |         delete_block(       [gcb '/f16InErrK1_D_Out']);
      |         add_block('built-in/Outport', [gcb '/f16InErrK1_D_Out'], 'Position', pos, 'Orientation', orient);
      | 
      |         pos = get_param(    [gcb '/f32Acc_Q_Out'], 'Position');
      |         orient = get_param( [gcb '/f32Acc_Q_Out'], 'Orientation');
      |         delete_block(       [gcb '/f32Acc_Q_Out']);
      |         add_block('built-in/Outport', [gcb '/f32Acc_Q_Out'], 'Position', pos, 'Orientation', orient);
      | 
      |         pos = get_param(    [gcb '/f16InErrK1_Q_Out'], 'Position');
      |         orient = get_param( [gcb '/f16InErrK1_Q_Out'], 'Orientation');
      |         delete_block(       [gcb '/f16InErrK1_Q_Out']);
      |         add_block('built-in/Outport', [gcb '/f16InErrK1_Q_Out'], 'Position', pos, 'Orientation', orient);
      | 
      | 
      |         set_param([gcb '/f16UDcBus'], 'Port', '1');
      |         set_param([gcb '/pIDQReq'], 'Port', '2');
      |         set_param([gcb '/pIDQFbck'], 'Port', '3');
      |         set_param([gcb '/f16ControllerPIrAWDOut_preset'], 'Port', '4');
      |         set_param([gcb '/f16ControllerPIrAWQOut_preset'], 'Port', '5');
      |         set_param([gcb '/f16CC1sc_D'], 'Port', '6');
      |         set_param([gcb '/f16CC2sc_D'], 'Port', '7');
      |         set_param([gcb '/u16NShift_D'], 'Port', '8');
      |         set_param([gcb '/f16CC1sc_Q'], 'Port', '9');
      |         set_param([gcb '/f16CC2sc_Q'], 'Port', '10');
      |         set_param([gcb '/u16NShift_Q'], 'Port', '11');
      |         set_param([gcb '/f32Acc_D'], 'Port', '12');
      |         set_param([gcb '/f16InErrK1_D'], 'Port', '13');
      |         set_param([gcb '/f32Acc_Q'], 'Port', '14');
      |         set_param([gcb '/f16InErrK1_Q'], 'Port', '15');
      | 
      |         set_param([gcb '/pUDQReq'], 'Port', '1');
      |         set_param([gcb '/f32Acc_D_Out'], 'Port', '2');
      |         set_param([gcb '/f16InErrK1_D_Out'], 'Port', '3');
      |         set_param([gcb '/f32Acc_Q_Out'], 'Port', '4');
      |         set_param([gcb '/f16InErrK1_Q_Out'], 'Port', '5');
      | 
      |         set_param(gcb,'MaskEnables',{'on','on','off','off','off','off','off','off'});
      | 
      |         if (posblk(4) - posblk(2)) < 400
      |           height = 400;
      |           set_param(gcb,'Position',[posblk(1), posblk(2), posblk(3), posblk(2)+height])
      |         end
      |     end
      | end
      settings: RTWSystemCode=Inline
      mask TypeOptions showStates: Hide (faster execution) | Show (allows debugging; connect feedback loops manually)
      mask Callback showStates:
      | maskStr = get_param(gcb,'showStates');
      | if strcmp(maskStr,'Hide (faster execution)'),
      |     set_param(gcb,'MaskEnables',{'on','on','on','on','on','on','on','on'});
      | else
      |     set_param(gcb,'MaskEnables',{'on','on','off','off','off','off','off','off'});
      | end
      mask TypeOptions resetStatesEnable: Pre-set according to the first set of inputs after reset | Clear to zero
      mask Display:
      | color('black');
      | pos = get_param(gcb, 'Position');
      | width = pos(3) - pos(1);
      | height = pos(4) - pos(2);
      | tX=width/2;
      | tY=height - 25;
      | color('black');
      | text(tX,tY, 'AMCLIB_CurrentLoop_F16', 'horizontalAlignment', 'center');
      | if showStates == 2
      |   color('red');
      |   text(tX,tY - 20, ['debugging mode' char(13) char(10) '(limited performance)'], 'horizontalAlignment', 'center');
      | end
  AMCLIB_FWSpeedLoop_F16 : Subsystem  TreatAsAtomicUnit=on  mask(AMCLIB_FWSpeedLoop_F16){showStates=Hide (faster execution), resetStatesEnable=Pre-set according to the first set of inputs after reset, showDebugOutputs=Hide, u16NSamplesW=0, u16NSamplesFW=0, f16PropGainQ=0, f16IntegGainQ=0, s16PropGainShiftQ=0, s16IntegGainShiftQ=0, f16LowerLimitQ=0, f16UpperLimitQ=0, f16PropGainFW=0, f16IntegGainFW=0, s16PropGainShiftFW=0, s16IntegGainShiftFW=0, f16LowerLimitFW=0, f16UpperLimitFW=0, f32RampUp=0, f32RampDown=0}
      mask prompts: showStates "Show internal states"; resetStatesEnable "Internal state after reset"; showDebugOutputs "Show debugging outputs"; u16NSamplesW "u16NSamplesW (velocity GDFLIB_FilterMA - recalculated smoothing factor)"; u16NSamplesFW "u16NSamplesFW (FW GDFLIB_FilterMA - recalculated smoothing factor)"; f16PropGainQ "f16PropGainQ (q-axis GFLIB_ControllerPIpAW - proportional gain)"; f16IntegGainQ "f16IntegGainQ (q-axis GFLIB_ControllerPIpAW - integral gain)"; s16PropGainShiftQ "s16PropGainShiftQ (q-axis GFLIB_ControllerPIpAW - scaling bitwise shift applied to the proportional gain)"; s16IntegGainShiftQ "s16IntegGainShiftQ (q-axis GFLIB_ControllerPIpAW - scaling bitwise shift applied to the integral gain)"; f16LowerLimitQ "f16LowerLimitQ (q-axis GFLIB_ControllerPIpAW - lower limit)"; f16UpperLimitQ "f16UpperLimitQ (q-axis GFLIB_ControllerPIpAW - upper limit)"; f16PropGainFW "f16PropGainFW (FW GFLIB_ControllerPIpAW - proportional gain)"; f16IntegGainFW "f16IntegGainFW (FW GFLIB_ControllerPIpAW - integral gain)"; s16PropGainShiftFW "s16PropGainShiftFW (FW GFLIB_ControllerPIpAW - scaling bitwise shift applied to the proportional gain)"; s16IntegGainShiftFW "s16IntegGainShiftFW (FW GFLIB_ControllerPIpAW - scaling bitwise shift applied to the integral gain)"; f16LowerLimitFW "f16LowerLimitFW (FW GFLIB_ControllerPIpAW - lower limit)"; f16UpperLimitFW "f16UpperLimitFW (FW GFLIB_ControllerPIpAW - upper limit)"; f32RampUp "f32RampUp (Ramp up increment coefficient)"; f32RampDown "f32RampDown (Ramp decrement coefficient)"
      mask help: Speed loop controller with Field Weakening capability for the PMSM field-oriented control algorithm in 16-bit fixed-point fractional implementation. This block supports re-initialization of the internal state during simulation. If the block is reset, the outputs of the MA filters, PI controllers, and the ramp will be aligned with the inputs f16FilterMAWOut_preset, f16FilterMAFWOut_preset, f16ControllerPIpAWQOut_preset, f16ControllerPIpAWFWOut_preset, and f32RampOut_preset. Refer to the AMMCLIB User's Guide for further details.
      mask init:
      | if ~evalin('base','exist(''tS8'',''var'')')
      |   if (2 ~= exist('SWLIBS_Typedefs.mat','file'))
      |       error('File SWLIBS_Typedefs.mat is not on the Matlab path. Please add the AMMCLIB "bam" folder in the Matlab Search Path.');
      |   else
      |       evalin('base', 'load(''SWLIBS_Typedefs.mat'')');
      |   end
      | end
      | if showStates == 1
      |     % hidden state variables
      |     if strcmp(get_param([gcb '/u16NSamplesW'], 'BlockType'), 'Inport')
      |         posblk = get_param(gcb, 'Position');
      | 
      |         pos = get_param(    [gcb, '/u16NSamplesW'], 'Position');
      |         orient = get_param( [gcb, '/u16NSamplesW'], 'Orientation');
      |         delete_block(       [gcb, '/u16NSamplesW']);
      |         add_block('built-in/Ground', [gcb, '/u16NSamplesW'], 'Position', pos, 'Orientation', orient);
      | 
      |         pos = get_param(    [gcb, '/u16NSamplesFW'], 'Position');
      |         orient = get_param( [gcb, '/u16NSamplesFW'], 'Orientation');
      |         delete_block(       [gcb, '/u16NSamplesFW']);
      |         add_block('built-in/Ground', [gcb, '/u16NSamplesFW'], 'Position', pos, 'Orientation', orient);
      | 
      |         pos = get_param(    [gcb, '/f16PropGainQ'], 'Position');
      |         orient = get_param( [gcb, '/f16PropGainQ'], 'Orientation');
      |         delete_block(       [gcb, '/f16PropGainQ']);
      |         add_block('built-in/Ground', [gcb, '/f16PropGainQ'], 'Position', pos, 'Orientation', orient);
      | 
      |         pos = get_param(    [gcb, '/f16IntegGainQ'], 'Position');
      |         orient = get_param( [gcb, '/f16IntegGainQ'], 'Orientation');
      |         delete_block(       [gcb, '/f16IntegGainQ']);
      |         add_block('built-in/Ground', [gcb, '/f16IntegGainQ'], 'Position', pos, 'Orientation', orient);
      | 
      |         pos = get_param(    [gcb, '/s16PropGainShiftQ'], 'Position');
      |         orient = get_param( [gcb, '/s16PropGainShiftQ'], 'Orientation');
      |         delete_block(       [gcb, '/s16PropGainShiftQ']);
      |         add_block('built-in/Ground', [gcb, '/s16PropGainShiftQ'], 'Position', pos, 'Orientation', orient);
      | 
      |         pos = get_param(    [gcb, '/s16IntegGainShiftQ'], 'Position');
      |         orient = get_param( [gcb, '/s16IntegGainShiftQ'], 'Orientation');
      |         delete_block(       [gcb, '/s16IntegGainShiftQ']);
      |         add_block('built-in/Ground', [gcb, '/s16IntegGainShiftQ'], 'Position', pos, 'Orientation', orient);
      | 
      |         pos = get_param(    [gcb, '/f16LowerLimitQ'], 'Position');
      |         orient = get_param( [gcb, '/f16LowerLimitQ'], 'Orientation');
      |         delete_block(       [gcb, '/f16LowerLimitQ']);
      |         add_block('built-in/Ground', [gcb, '/f16LowerLimitQ'], 'Position', pos, 'Orientation', orient);
      | 
      |         pos = get_param(    [gcb, '/f16UpperLimitQ'], 'Position');
      |         orient = get_param( [gcb, '/f16UpperLimitQ'], 'Orientation');
      |         delete_block(       [gcb, '/f16UpperLimitQ']);
      |         add_block('built-in/Ground', [gcb, '/f16UpperLimitQ'], 'Position', pos, 'Orientation', orient);
      | 
      |         pos = get_param(    [gcb, '/f16PropGainFW'], 'Position');
      |         orient = get_param( [gcb, '/f16PropGainFW'], 'Orientation');
      |         delete_block(       [gcb, '/f16PropGainFW']);
      |         add_block('built-in/Ground', [gcb, '/f16PropGainFW'], 'Position', pos, 'Orientation', orient);
      | 
      |         pos = get_param(    [gcb, '/f16IntegGainFW'], 'Position');
      |         orient = get_param( [gcb, '/f16IntegGainFW'], 'Orientation');
      |         delete_block(       [gcb, '/f16IntegGainFW']);
      |         add_block('built-in/Ground', [gcb, '/f16IntegGainFW'], 'Position', pos, 'Orientation', orient);
      | 
      |         pos = get_param(    [gcb, '/s16PropGainShiftFW'], 'Position');
      |         orient = get_param( [gcb, '/s16PropGainShiftFW'], 'Orientation');
      |         delete_block(       [gcb, '/s16PropGainShiftFW']);
      |         add_block('built-in/Ground', [gcb, '/s16PropGainShiftFW'], 'Position', pos, 'Orientation', orient);
      | 
      |         pos = get_param(    [gcb, '/s16IntegGainShiftFW'], 'Position');
      |         orient = get_param( [gcb, '/s16IntegGainShiftFW'], 'Orientation');
      |         delete_block(       [gcb, '/s16IntegGainShiftFW']);
      |         add_block('built-in/Ground', [gcb, '/s16IntegGainShiftFW'], 'Position', pos, 'Orientation', orient);
      | 
      |         pos = get_param(    [gcb, '/f16LowerLimitFW'], 'Position');
      |         orient = get_param( [gcb, '/f16LowerLimitFW'], 'Orientation');
      |         delete_block(       [gcb, '/f16LowerLimitFW']);
      |         add_block('built-in/Ground', [gcb, '/f16LowerLimitFW'], 'Position', pos, 'Orientation', orient);
      | 
      |         pos = get_param(    [gcb, '/f16UpperLimitFW'], 'Position');
      |         orient = get_param( [gcb, '/f16UpperLimitFW'], 'Orientation');
      |         delete_block(       [gcb, '/f16UpperLimitFW']);
      |         add_block('built-in/Ground', [gcb, '/f16UpperLimitFW'], 'Position', pos, 'Orientation', orient);
      | 
      |         pos = get_param(    [gcb, '/f32RampUp'], 'Position');
      |         orient = get_param( [gcb, '/f32RampUp'], 'Orientation');
      |         delete_block(       [gcb, '/f32RampUp']);
      |         add_block('built-in/Ground', [gcb, '/f32RampUp'], 'Position', pos, 'Orientation', orient);
      | 
      |         pos = get_param(    [gcb, '/f32RampDown'], 'Position');
      |         orient = get_param( [gcb, '/f32RampDown'], 'Orientation');
      |         delete_block(       [gcb, '/f32RampDown']);
      |         add_block('built-in/Ground', [gcb, '/f32RampDown'], 'Position', pos, 'Orientation', orient);
      | 
      |         pos = get_param(    [gcb, '/f16IQReqK_1'], 'Position');
      |         orient = get_param( [gcb, '/f16IQReqK_1'], 'Orientation');
      |         delete_block(       [gcb, '/f16IQReqK_1']);
      |         add_block('built-in/Ground', [gcb, '/f16IQReqK_1'], 'Position', pos, 'Orientation', orient);
      | 
      |         pos = get_param(    [gcb, '/f32AccW'], 'Position');
      |         orient = get_param( [gcb, '/f32AccW'], 'Orientation');
      |         delete_block(       [gcb, '/f32AccW']);
      |         add_block('built-in/Ground', [gcb, '/f32AccW'], 'Position', pos, 'Orientation', orient);
      | 
      |         pos = get_param(    [gcb, '/f32AccFW'], 'Position');
      |         orient = get_param( [gcb, '/f32AccFW'], 'Orientation');
      |         delete_block(       [gcb, '/f32AccFW']);
      |         add_block('built-in/Ground', [gcb, '/f32AccFW'], 'Position', pos, 'Orientation', orient);
      | 
      |         pos = get_param(    [gcb, '/f32IntegPartK_1Q'], 'Position');
      |         orient = get_param( [gcb, '/f32IntegPartK_1Q'], 'Orientation');
      |         delete_block(       [gcb, '/f32IntegPartK_1Q']);
      |         add_block('built-in/Ground', [gcb, '/f32IntegPartK_1Q'], 'Position', pos, 'Orientation', orient);
      | 
      |         pos = get_param(    [gcb, '/f16InK_1Q'], 'Position');
      |         orient = get_param( [gcb, '/f16InK_1Q'], 'Orientation');
      |         delete_block(       [gcb, '/f16InK_1Q']);
      |         add_block('built-in/Ground', [gcb, '/f16InK_1Q'], 'Position', pos, 'Orientation', orient);
      | 
      |         pos = get_param(    [gcb, '/f32IntegPartK_1FW'], 'Position');
      |         orient = get_param( [gcb, '/f32IntegPartK_1FW'], 'Orientation');
      |         delete_block(       [gcb, '/f32IntegPartK_1FW']);
      |         add_block('built-in/Ground', [gcb, '/f32IntegPartK_1FW'], 'Position', pos, 'Orientation', orient);
      | 
      |         pos = get_param(    [gcb, '/f16InK_1FW'], 'Position');
      |         orient = get_param( [gcb, '/f16InK_1FW'], 'Orientation');
      |         delete_block(       [gcb, '/f16InK_1FW']);
      |         add_block('built-in/Ground', [gcb, '/f16InK_1FW'], 'Position', pos, 'Orientation', orient);
      | 
      |         pos = get_param(    [gcb, '/f32State'], 'Position');
      |         orient = get_param( [gcb, '/f32State'], 'Orientation');
      |         delete_block(       [gcb, '/f32State']);
      |         add_block('built-in/Ground', [gcb, '/f32State'], 'Position', pos, 'Orientation', orient);
      | 
      | 
      |         pos = get_param(    [gcb '/f32AccW_Out'], 'Position');
      |         orient = get_param( [gcb '/f32AccW_Out'], 'Orientation');
      |         delete_block(       [gcb '/f32AccW_Out']);
      |         add_block('built-in/Terminator', [gcb '/f32AccW_Out'], 'Position', pos, 'Orientation', orient);
      | 
      |         pos = get_param(    [gcb '/f32AccFW_Out'], 'Position');
      |         orient = get_param( [gcb '/f32AccFW_Out'], 'Orientation');
      |         delete_block(       [gcb '/f32AccFW_Out']);
      |         add_block('built-in/Terminator', [gcb '/f32AccFW_Out'], 'Position', pos, 'Orientation', orient);
      | 
      |         pos = get_param(    [gcb '/f32IntegPartK_1Q_Out'], 'Position');
      |         orient = get_param( [gcb '/f32IntegPartK_1Q_Out'], 'Orientation');
      |         delete_block(       [gcb '/f32IntegPartK_1Q_Out']);
      |         add_block('built-in/Terminator', [gcb '/f32IntegPartK_1Q_Out'], 'Position', pos, 'Orientation', orient);
      | 
      |         pos = get_param(    [gcb '/f16InK_1Q_Out'], 'Position');
      |         orient = get_param( [gcb '/f16InK_1Q_Out'], 'Orientation');
      |         delete_block(       [gcb '/f16InK_1Q_Out']);
      |         add_block('built-in/Terminator', [gcb '/f16InK_1Q_Out'], 'Position', pos, 'Orientation', orient);
      | 
      |         pos = get_param(    [gcb '/f32IntegPartK_1FW_Out'], 'Position');
      |         orient = get_param( [gcb '/f32IntegPartK_1FW_Out'], 'Orientation');
      |         delete_block(       [gcb '/f32IntegPartK_1FW_Out']);
      |         add_block('built-in/Terminator', [gcb '/f32IntegPartK_1FW_Out'], 'Position', pos, 'Orientation', orient);
      | 
      |         pos = get_param(    [gcb '/f16InK_1FW_Out'], 'Position');
      |         orient = get_param( [gcb '/f16InK_1FW_Out'], 'Orientation');
      |         delete_block(       [gcb '/f16InK_1FW_Out']);
      |         add_block('built-in/Terminator', [gcb '/f16InK_1FW_Out'], 'Position', pos, 'Orientation', orient);
      | 
      |         pos = get_param(    [gcb '/f32State_Out'], 'Position');
      |         orient = get_param( [gcb '/f32State_Out'], 'Orientation');
      |         delete_block(       [gcb '/f32State_Out']);
      |         add_block('built-in/Terminator', [gcb '/f32State_Out'], 'Position', pos, 'Orientation', orient);
      | 
      | 
      |         if strcmp(get_param([gcb '/f16WReqFilt'], 'BlockType'), 'Outport')
      |             pos = get_param(    [gcb '/f16WReqFilt'], 'Position');
      |             orient = get_param( [gcb '/f16WReqFilt'], 'Orientation');
      |             delete_block(       [gcb '/f16WReqFilt']);
      |             add_block('built-in/Terminator', [gcb '/f16WReqFilt'], 'Position', pos, 'Orientation', orient);
      | 
      |             pos = get_param(    [gcb '/f16WErr'], 'Position');
      |             orient = get_param( [gcb '/f16WErr'], 'Orientation');
      |             delete_block(       [gcb '/f16WErr']);
      |             add_block('built-in/Terminator', [gcb '/f16WErr'], 'Position', pos, 'Orientation', orient);
      | 
      |             pos = get_param(    [gcb '/f16IDQReqAmp'], 'Position');
      |             orient = get_param( [gcb '/f16IDQReqAmp'], 'Orientation');
      |             delete_block(       [gcb '/f16IDQReqAmp']);
      |             add_block('built-in/Terminator', [gcb '/f16IDQReqAmp'], 'Position', pos, 'Orientation', orient);
      | 
      |             pos = get_param(    [gcb '/f16WFbckFilt'], 'Position');
      |             orient = get_param( [gcb '/f16WFbckFilt'], 'Orientation');
      |             delete_block(       [gcb '/f16WFbckFilt']);
      |             add_block('built-in/Terminator', [gcb '/f16WFbckFilt'], 'Position', pos, 'Orientation', orient);
      | 
      |             pos = get_param(    [gcb '/f16IQErrSign'], 'Position');
      |             orient = get_param( [gcb '/f16IQErrSign'], 'Orientation');
      |             delete_block(       [gcb '/f16IQErrSign']);
      |             add_block('built-in/Terminator', [gcb '/f16IQErrSign'], 'Position', pos, 'Orientation', orient);
      | 
      |             pos = get_param(    [gcb '/f16IQErr'], 'Position');
      |             orient = get_param( [gcb '/f16IQErr'], 'Orientation');
      |             delete_block(       [gcb '/f16IQErr']);
      |             add_block('built-in/Terminator', [gcb '/f16IQErr'], 'Position', pos, 'Orientation', orient);
      | 
      |             pos = get_param(    [gcb '/f16FWErr'], 'Position');
      |             orient = get_param( [gcb '/f16FWErr'], 'Orientation');
      |             delete_block(       [gcb '/f16FWErr']);
      |             add_block('built-in/Terminator', [gcb '/f16FWErr'], 'Position', pos, 'Orientation', orient);
      | 
      |             pos = get_param(    [gcb '/f16UQErr'], 'Position');
      |             orient = get_param( [gcb '/f16UQErr'], 'Orientation');
      |             delete_block(       [gcb '/f16UQErr']);
      |             add_block('built-in/Terminator', [gcb '/f16UQErr'], 'Position', pos, 'Orientation', orient);
      | 
      |             pos = get_param(    [gcb '/f16FWErrFilt'], 'Position');
      |             orient = get_param( [gcb '/f16FWErrFilt'], 'Orientation');
      |             delete_block(       [gcb '/f16FWErrFilt']);
      |             add_block('built-in/Terminator', [gcb '/f16FWErrFilt'], 'Position', pos, 'Orientation', orient);
      | 
      |             pos = get_param(    [gcb '/f16FWAngle'], 'Position');
      |             orient = get_param( [gcb '/f16FWAngle'], 'Orientation');
      |             delete_block(       [gcb '/f16FWAngle']);
      |             add_block('built-in/Terminator', [gcb '/f16FWAngle'], 'Position', pos, 'Orientation', orient);
      | 
      |             pos = get_param(    [gcb '/f16FWSin'], 'Position');
      |             orient = get_param( [gcb '/f16FWSin'], 'Orientation');
      |             delete_block(       [gcb '/f16FWSin']);
      |             add_block('built-in/Terminator', [gcb '/f16FWSin'], 'Position', pos, 'Orientation', orient);
      | 
      |             pos = get_param(    [gcb '/f16FWCos'], 'Position');
      |             orient = get_param( [gcb '/f16FWCos'], 'Orientation');
      |             delete_block(       [gcb '/f16FWCos']);
      |             add_block('built-in/Terminator', [gcb '/f16FWCos'], 'Position', pos, 'Orientation', orient);
      | 
      |         end
      | 
      |         set_param([gcb '/f16VelocityReq'], 'Port', '1');
      |         set_param([gcb '/f16VelocityFbck'], 'Port', '2');
      |         set_param([gcb '/f16IQFbck'], 'Port', '3');
      |         set_param([gcb '/f16UQReq'], 'Port', '4');
      |         set_param([gcb '/f16UQLim'], 'Port', '5');
      |         set_param([gcb '/f16FilterMAWOut_preset'], 'Port', '6');
      |         set_param([gcb '/f16FilterMAFWOut_preset'], 'Port', '7');
      |         set_param([gcb '/f16ControllerPIpAWQOut_preset'], 'Port', '8');
      |         set_param([gcb '/f16ControllerPIpAWFWOut_preset'], 'Port', '9');
      |         set_param([gcb '/f32RampOut_preset'], 'Port', '10');
      | 
      |         set_param([gcb '/pIDQReq'], 'Port', '1');
      |         set_param([gcb '/u16LimitFlagQ'], 'Port', '2');
      |         set_param([gcb '/u16LimitFlagFW'], 'Port', '3');
      | 
      |         set_param(gcb,'MaskEnables',{'on','on','off','on','on','on','on','on','on','on','on','on','on','on','on','on','on','on','on'});
      | 
      |         if (posblk(4) - posblk(2)) > 275
      |           height = 275;
      |           set_param(gcb,'Position',[posblk(1), posblk(2), posblk(3), posblk(2)+height])
      |         end
      |     end
      | else
      |     % shown state variables
      |     if strcmp(get_param([gcb '/u16NSamplesW'], 'BlockType'), 'Ground')
      |         posblk = get_param(gcb, 'Position');
      | 
      |         pos = get_param(    [gcb, '/u16NSamplesW'], 'Position');
      |         orient = get_param( [gcb, '/u16NSamplesW'], 'Orientation');
      |         delete_block(       [gcb, '/u16NSamplesW']);
      |         add_block('built-in/Inport', [gcb, '/u16NSamplesW'], 'Position', pos, 'Orientation', orient, 'OutDataTypeStr', 'uint16');
      | 
      |         pos = get_param(    [gcb, '/u16NSamplesFW'], 'Position');
      |         orient = get_param( [gcb, '/u16NSamplesFW'], 'Orientation');
      |         delete_block(       [gcb, '/u16NSamplesFW']);
      |         add_block('built-in/Inport', [gcb, '/u16NSamplesFW'], 'Position', pos, 'Orientation', orient, 'OutDataTypeStr', 'uint16');
      | 
      |         pos = get_param(    [gcb, '/f16PropGainQ'], 'Position');
      |         orient = get_param( [gcb, '/f16PropGainQ'], 'Orientation');
      |         delete_block(       [gcb, '/f16PropGainQ']);
      |         add_block('built-in/Inport', [gcb, '/f16PropGainQ'], 'Position', pos, 'Orientation', orient, 'OutDataTypeStr', 'int16');
      | 
      |         pos = get_param(    [gcb, '/f16IntegGainQ'], 'Position');
      |         orient = get_param( [gcb, '/f16IntegGainQ'], 'Orientation');
      |         delete_block(       [gcb, '/f16IntegGainQ']);
      |         add_block('built-in/Inport', [gcb, '/f16IntegGainQ'], 'Position', pos, 'Orientation', orient, 'OutDataTypeStr', 'int16');
      | 
      |         pos = get_param(    [gcb, '/s16PropGainShiftQ'], 'Position');
      |         orient = get_param( [gcb, '/s16PropGainShiftQ'], 'Orientation');
      |         delete_block(       [gcb, '/s16PropGainShiftQ']);
      |         add_block('built-in/Inport', [gcb, '/s16PropGainShiftQ'], 'Position', pos, 'Orientation', orient, 'OutDataTypeStr', 'int16');
      | 
      |         pos = get_param(    [gcb, '/s16IntegGainShiftQ'], 'Position');
      |         orient = get_param( [gcb, '/s16IntegGainShiftQ'], 'Orientation');
      |         delete_block(       [gcb, '/s16IntegGainShiftQ']);
      |         add_block('built-in/Inport', [gcb, '/s16IntegGainShiftQ'], 'Position', pos, 'Orientation', orient, 'OutDataTypeStr', 'int16');
      | 
      |         pos = get_param(    [gcb, '/f16LowerLimitQ'], 'Position');
      |         orient = get_param( [gcb, '/f16LowerLimitQ'], 'Orientation');
      |         delete_block(       [gcb, '/f16LowerLimitQ']);
      |         add_block('built-in/Inport', [gcb, '/f16LowerLimitQ'], 'Position', pos, 'Orientation', orient, 'OutDataTypeStr', 'int16');
      | 
      |         pos = get_param(    [gcb, '/f16UpperLimitQ'], 'Position');
      |         orient = get_param( [gcb, '/f16UpperLimitQ'], 'Orientation');
      |         delete_block(       [gcb, '/f16UpperLimitQ']);
      |         add_block('built-in/Inport', [gcb, '/f16UpperLimitQ'], 'Position', pos, 'Orientation', orient, 'OutDataTypeStr', 'int16');
      | 
      |         pos = get_param(    [gcb, '/f16PropGainFW'], 'Position');
      |         orient = get_param( [gcb, '/f16PropGainFW'], 'Orientation');
      |         delete_block(       [gcb, '/f16PropGainFW']);
      |         add_block('built-in/Inport', [gcb, '/f16PropGainFW'], 'Position', pos, 'Orientation', orient, 'OutDataTypeStr', 'int16');
      | 
      |         pos = get_param(    [gcb, '/f16IntegGainFW'], 'Position');
      |         orient = get_param( [gcb, '/f16IntegGainFW'], 'Orientation');
      |         delete_block(       [gcb, '/f16IntegGainFW']);
      |         add_block('built-in/Inport', [gcb, '/f16IntegGainFW'], 'Position', pos, 'Orientation', orient, 'OutDataTypeStr', 'int16');
      | 
      |         pos = get_param(    [gcb, '/s16PropGainShiftFW'], 'Position');
      |         orient = get_param( [gcb, '/s16PropGainShiftFW'], 'Orientation');
      |         delete_block(       [gcb, '/s16PropGainShiftFW']);
      |         add_block('built-in/Inport', [gcb, '/s16PropGainShiftFW'], 'Position', pos, 'Orientation', orient, 'OutDataTypeStr', 'int16');
      | 
      |         pos = get_param(    [gcb, '/s16IntegGainShiftFW'], 'Position');
      |         orient = get_param( [gcb, '/s16IntegGainShiftFW'], 'Orientation');
      |         delete_block(       [gcb, '/s16IntegGainShiftFW']);
      |         add_block('built-in/Inport', [gcb, '/s16IntegGainShiftFW'], 'Position', pos, 'Orientation', orient, 'OutDataTypeStr', 'int16');
      | 
      |         pos = get_param(    [gcb, '/f16LowerLimitFW'], 'Position');
      |         orient = get_param( [gcb, '/f16LowerLimitFW'], 'Orientation');
      |         delete_block(       [gcb, '/f16LowerLimitFW']);
      |         add_block('built-in/Inport', [gcb, '/f16LowerLimitFW'], 'Position', pos, 'Orientation', orient, 'OutDataTypeStr', 'int16');
      | 
      |         pos = get_param(    [gcb, '/f16UpperLimitFW'], 'Position');
      |         orient = get_param( [gcb, '/f16UpperLimitFW'], 'Orientation');
      |         delete_block(       [gcb, '/f16UpperLimitFW']);
      |         add_block('built-in/Inport', [gcb, '/f16UpperLimitFW'], 'Position', pos, 'Orientation', orient, 'OutDataTypeStr', 'int16');
      | 
      |         pos = get_param(    [gcb, '/f32RampUp'], 'Position');
      |         orient = get_param( [gcb, '/f32RampUp'], 'Orientation');
      |         delete_block(       [gcb, '/f32RampUp']);
      |         add_block('built-in/Inport', [gcb, '/f32RampUp'], 'Position', pos, 'Orientation', orient, 'OutDataTypeStr', 'int32');
      | 
      |         pos = get_param(    [gcb, '/f32RampDown'], 'Position');
      |         orient = get_param( [gcb, '/f32RampDown'], 'Orientation');
      |         delete_block(       [gcb, '/f32RampDown']);
      |         add_block('built-in/Inport', [gcb, '/f32RampDown'], 'Position', pos, 'Orientation', orient, 'OutDataTypeStr', 'int32');
      | 
      |         pos = get_param(    [gcb, '/f16IQReqK_1'], 'Position');
      |         orient = get_param( [gcb, '/f16IQReqK_1'], 'Orientation');
      |         delete_block(       [gcb, '/f16IQReqK_1']);
      |         add_block('built-in/Inport', [gcb, '/f16IQReqK_1'], 'Position', pos, 'Orientation', orient, 'OutDataTypeStr', 'int16');
      | 
      |         pos = get_param(    [gcb, '/f32AccW'], 'Position');
      |         orient = get_param( [gcb, '/f32AccW'], 'Orientation');
      |         delete_block(       [gcb, '/f32AccW']);
      |         add_block('built-in/Inport', [gcb, '/f32AccW'], 'Position', pos, 'Orientation', orient, 'OutDataTypeStr', 'int32');
      | 
      |         pos = get_param(    [gcb, '/f32AccFW'], 'Position');
      |         orient = get_param( [gcb, '/f32AccFW'], 'Orientation');
      |         delete_block(       [gcb, '/f32AccFW']);
      |         add_block('built-in/Inport', [gcb, '/f32AccFW'], 'Position', pos, 'Orientation', orient, 'OutDataTypeStr', 'int32');
      | 
      |         pos = get_param(    [gcb, '/f32IntegPartK_1Q'], 'Position');
      |         orient = get_param( [gcb, '/f32IntegPartK_1Q'], 'Orientation');
      |         delete_block(       [gcb, '/f32IntegPartK_1Q']);
      |         add_block('built-in/Inport', [gcb, '/f32IntegPartK_1Q'], 'Position', pos, 'Orientation', orient, 'OutDataTypeStr', 'int32');
      | 
      |         pos = get_param(    [gcb, '/f16InK_1Q'], 'Position');
      |         orient = get_param( [gcb, '/f16InK_1Q'], 'Orientation');
      |         delete_block(       [gcb, '/f16InK_1Q']);
      |         add_block('built-in/Inport', [gcb, '/f16InK_1Q'], 'Position', pos, 'Orientation', orient, 'OutDataTypeStr', 'int16');
      | 
      |         pos = get_param(    [gcb, '/f32IntegPartK_1FW'], 'Position');
      |         orient = get_param( [gcb, '/f32IntegPartK_1FW'], 'Orientation');
      |         delete_block(       [gcb, '/f32IntegPartK_1FW']);
      |         add_block('built-in/Inport', [gcb, '/f32IntegPartK_1FW'], 'Position', pos, 'Orientation', orient, 'OutDataTypeStr', 'int32');
      | 
      |         pos = get_param(    [gcb, '/f16InK_1FW'], 'Position');
      |         orient = get_param( [gcb, '/f16InK_1FW'], 'Orientation');
      |         delete_block(       [gcb, '/f16InK_1FW']);
      |         add_block('built-in/Inport', [gcb, '/f16InK_1FW'], 'Position', pos, 'Orientation', orient, 'OutDataTypeStr', 'int16');
      | 
      |         pos = get_param(    [gcb, '/f32State'], 'Position');
      |         orient = get_param( [gcb, '/f32State'], 'Orientation');
      |         delete_block(       [gcb, '/f32State']);
      |         add_block('built-in/Inport', [gcb, '/f32State'], 'Position', pos, 'Orientation', orient, 'OutDataTypeStr', 'int32');
      | 
      | 
      |         pos = get_param(    [gcb '/f32AccW_Out'], 'Position');
      |         orient = get_param( [gcb '/f32AccW_Out'], 'Orientation');
      |         delete_block(       [gcb '/f32AccW_Out']);
      |         add_block('built-in/Outport', [gcb '/f32AccW_Out'], 'Position', pos, 'Orientation', orient);
      | 
      |         pos = get_param(    [gcb '/f32AccFW_Out'], 'Position');
      |         orient = get_param( [gcb '/f32AccFW_Out'], 'Orientation');
      |         delete_block(       [gcb '/f32AccFW_Out']);
      |         add_block('built-in/Outport', [gcb '/f32AccFW_Out'], 'Position', pos, 'Orientation', orient);
      | 
      |         pos = get_param(    [gcb '/f32IntegPartK_1Q_Out'], 'Position');
      |         orient = get_param( [gcb '/f32IntegPartK_1Q_Out'], 'Orientation');
      |         delete_block(       [gcb '/f32IntegPartK_1Q_Out']);
      |         add_block('built-in/Outport', [gcb '/f32IntegPartK_1Q_Out'], 'Position', pos, 'Orientation', orient);
      | 
      |         pos = get_param(    [gcb '/f16InK_1Q_Out'], 'Position');
      |         orient = get_param( [gcb '/f16InK_1Q_Out'], 'Orientation');
      |         delete_block(       [gcb '/f16InK_1Q_Out']);
      |         add_block('built-in/Outport', [gcb '/f16InK_1Q_Out'], 'Position', pos, 'Orientation', orient);
      | 
      |         pos = get_param(    [gcb '/f32IntegPartK_1FW_Out'], 'Position');
      |         orient = get_param( [gcb '/f32IntegPartK_1FW_Out'], 'Orientation');
      |         delete_block(       [gcb '/f32IntegPartK_1FW_Out']);
      |         add_block('built-in/Outport', [gcb '/f32IntegPartK_1FW_Out'], 'Position', pos, 'Orientation', orient);
      | 
      |         pos = get_param(    [gcb '/f16InK_1FW_Out'], 'Position');
      |         orient = get_param( [gcb '/f16InK_1FW_Out'], 'Orientation');
      |         delete_block(       [gcb '/f16InK_1FW_Out']);
      |         add_block('built-in/Outport', [gcb '/f16InK_1FW_Out'], 'Position', pos, 'Orientation', orient);
      | 
      |         pos = get_param(    [gcb '/f32State_Out'], 'Position');
      |         orient = get_param( [gcb '/f32State_Out'], 'Orientation');
      |         delete_block(       [gcb '/f32State_Out']);
      |         add_block('built-in/Outport', [gcb '/f32State_Out'], 'Position', pos, 'Orientation', orient);
      | 
      | 
      |         if (showDebugOutputs == 2) && (strcmp(get_param([gcb '/f16WReqFilt'], 'BlockType'), 'Terminator'))
      |             pos = get_param(    [gcb '/f16WReqFilt'], 'Position');
      |             orient = get_param( [gcb '/f16WReqFilt'], 'Orientation');
      |             delete_block(       [gcb '/f16WReqFilt']);
      |             add_block('built-in/Outport', [gcb '/f16WReqFilt'], 'Position', pos, 'Orientation', orient);
      | 
      |             pos = get_param(    [gcb '/f16WErr'], 'Position');
      |             orient = get_param( [gcb '/f16WErr'], 'Orientation');
      |             delete_block(       [gcb '/f16WErr']);
      |             add_block('built-in/Outport', [gcb '/f16WErr'], 'Position', pos, 'Orientation', orient);
      | 
      |             pos = get_param(    [gcb '/f16IDQReqAmp'], 'Position');
      |             orient = get_param( [gcb '/f16IDQReqAmp'], 'Orientation');
      |             delete_block(       [gcb '/f16IDQReqAmp']);
      |             add_block('built-in/Outport', [gcb '/f16IDQReqAmp'], 'Position', pos, 'Orientation', orient);
      | 
      |             pos = get_param(    [gcb '/f16WFbckFilt'], 'Position');
      |             orient = get_param( [gcb '/f16WFbckFilt'], 'Orientation');
      |             delete_block(       [gcb '/f16WFbckFilt']);
      |             add_block('built-in/Outport', [gcb '/f16WFbckFilt'], 'Position', pos, 'Orientation', orient);
      | 
      |             pos = get_param(    [gcb '/f16IQErrSign'], 'Position');
      |             orient = get_param( [gcb '/f16IQErrSign'], 'Orientation');
      |             delete_block(       [gcb '/f16IQErrSign']);
      |             add_block('built-in/Outport', [gcb '/f16IQErrSign'], 'Position', pos, 'Orientation', orient);
      | 
      |             pos = get_param(    [gcb '/f16IQErr'], 'Position');
      |             orient = get_param( [gcb '/f16IQErr'], 'Orientation');
      |             delete_block(       [gcb '/f16IQErr']);
      |             add_block('built-in/Outport', [gcb '/f16IQErr'], 'Position', pos, 'Orientation', orient);
      | 
      |             pos = get_param(    [gcb '/f16FWErr'], 'Position');
      |             orient = get_param( [gcb '/f16FWErr'], 'Orientation');
      |             delete_block(       [gcb '/f16FWErr']);
      |             add_block('built-in/Outport', [gcb '/f16FWErr'], 'Position', pos, 'Orientation', orient);
      | 
      |             pos = get_param(    [gcb '/f16UQErr'], 'Position');
      |             orient = get_param( [gcb '/f16UQErr'], 'Orientation');
      |             delete_block(       [gcb '/f16UQErr']);
      |             add_block('built-in/Outport', [gcb '/f16UQErr'], 'Position', pos, 'Orientation', orient);
      | 
      |             pos = get_param(    [gcb '/f16FWErrFilt'], 'Position');
      |             orient = get_param( [gcb '/f16FWErrFilt'], 'Orientation');
      |             delete_block(       [gcb '/f16FWErrFilt']);
      |             add_block('built-in/Outport', [gcb '/f16FWErrFilt'], 'Position', pos, 'Orientation', orient);
      | 
      |             pos = get_param(    [gcb '/f16FWAngle'], 'Position');
      |             orient = get_param( [gcb '/f16FWAngle'], 'Orientation');
      |             delete_block(       [gcb '/f16FWAngle']);
      |             add_block('built-in/Outport', [gcb '/f16FWAngle'], 'Position', pos, 'Orientation', orient);
      | 
      |             pos = get_param(    [gcb '/f16FWSin'], 'Position');
      |             orient = get_param( [gcb '/f16FWSin'], 'Orientation');
      |             delete_block(       [gcb '/f16FWSin']);
      |             add_block('built-in/Outport', [gcb '/f16FWSin'], 'Position', pos, 'Orientation', orient);
      | 
      |             pos = get_param(    [gcb '/f16FWCos'], 'Position');
      |             orient = get_param( [gcb '/f16FWCos'], 'Orientation');
      |             delete_block(       [gcb '/f16FWCos']);
      |             add_block('built-in/Outport', [gcb '/f16FWCos'], 'Position', pos, 'Orientation', orient);
      | 
      |         end
      | 
      |         set_param([gcb '/f16VelocityReq'], 'Port', '1');
      |         set_param([gcb '/f16VelocityFbck'], 'Port', '2');
      |         set_param([gcb '/f16IQFbck'], 'Port', '3');
      |         set_param([gcb '/f16UQReq'], 'Port', '4');
      |         set_param([gcb '/f16UQLim'], 'Port', '5');
      |         set_param([gcb '/f16FilterMAWOut_preset'], 'Port', '6');
      |         set_param([gcb '/f16FilterMAFWOut_preset'], 'Port', '7');
      |         set_param([gcb '/f16ControllerPIpAWQOut_preset'], 'Port', '8');
      |         set_param([gcb '/f16ControllerPIpAWFWOut_preset'], 'Port', '9');
      |         set_param([gcb '/f32RampOut_preset'], 'Port', '10');
      |         set_param([gcb '/u16NSamplesW'], 'Port', '11');
      |         set_param([gcb '/u16NSamplesFW'], 'Port', '12');
      |         set_param([gcb '/f16PropGainQ'], 'Port', '13');
      |         set_param([gcb '/f16IntegGainQ'], 'Port', '14');
      |         set_param([gcb '/s16PropGainShiftQ'], 'Port', '15');
      |         set_param([gcb '/s16IntegGainShiftQ'], 'Port', '16');
      |         set_param([gcb '/f16LowerLimitQ'], 'Port', '17');
      |         set_param([gcb '/f16UpperLimitQ'], 'Port', '18');
      |         set_param([gcb '/f16PropGainFW'], 'Port', '19');
      |         set_param([gcb '/f16IntegGainFW'], 'Port', '20');
      |         set_param([gcb '/s16PropGainShiftFW'], 'Port', '21');
      |         set_param([gcb '/s16IntegGainShiftFW'], 'Port', '22');
      |         set_param([gcb '/f16LowerLimitFW'], 'Port', '23');
      |         set_param([gcb '/f16UpperLimitFW'], 'Port', '24');
      |         set_param([gcb '/f32RampUp'], 'Port', '25');
      |         set_param([gcb '/f32RampDown'], 'Port', '26');
      |         set_param([gcb '/f16IQReqK_1'], 'Port', '27');
      |         set_param([gcb '/f32AccW'], 'Port', '28');
      |         set_param([gcb '/f32AccFW'], 'Port', '29');
      |         set_param([gcb '/f32IntegPartK_1Q'], 'Port', '30');
      |         set_param([gcb '/f16InK_1Q'], 'Port', '31');
      |         set_param([gcb '/f32IntegPartK_1FW'], 'Port', '32');
      |         set_param([gcb '/f16InK_1FW'], 'Port', '33');
      |         set_param([gcb '/f32State'], 'Port', '34');
      | 
      |         if (showDebugOutputs == 2)
      |             set_param([gcb '/pIDQReq'], 'Port', '1');
      |             set_param([gcb '/u16LimitFlagQ'], 'Port', '2');
      |             set_param([gcb '/u16LimitFlagFW'], 'Port', '3');
      |             set_param([gcb '/f16WReqFilt'], 'Port', '4');
      |             set_param([gcb '/f16WErr'], 'Port', '5');
      |             set_param([gcb '/f16IDQReqAmp'], 'Port', '6');
      |             set_param([gcb '/f16WFbckFilt'], 'Port', '7');
      |             set_param([gcb '/f16IQErrSign'], 'Port', '8');
      |             set_param([gcb '/f16IQErr'], 'Port', '9');
      |             set_param([gcb '/f16FWErr'], 'Port', '10');
      |             set_param([gcb '/f16UQErr'], 'Port', '11');
      |             set_param([gcb '/f16FWErrFilt'], 'Port', '12');
      |             set_param([gcb '/f16FWAngle'], 'Port', '13');
      |             set_param([gcb '/f16FWSin'], 'Port', '14');
      |             set_param([gcb '/f16FWCos'], 'Port', '15');
      |             set_param([gcb '/f32AccW_Out'], 'Port', '16');
      |             set_param([gcb '/f32AccFW_Out'], 'Port', '17');
      |             set_param([gcb '/f32IntegPartK_1Q_Out'], 'Port', '18');
      |             set_param([gcb '/f16InK_1Q_Out'], 'Port', '19');
      |             set_param([gcb '/f32IntegPartK_1FW_Out'], 'Port', '20');
      |             set_param([gcb '/f16InK_1FW_Out'], 'Port', '21');
      |             set_param([gcb '/f32State_Out'], 'Port', '22');
      |         else
      |             set_param([gcb '/pIDQReq'], 'Port', '1');
      |             set_param([gcb '/u16LimitFlagQ'], 'Port', '2');
      |             set_param([gcb '/u16LimitFlagFW'], 'Port', '3');
      |             set_param([gcb '/f32AccW_Out'], 'Port', '4');
      |             set_param([gcb '/f32AccFW_Out'], 'Port', '5');
      |             set_param([gcb '/f32IntegPartK_1Q_Out'], 'Port', '6');
      |             set_param([gcb '/f16InK_1Q_Out'], 'Port', '7');
      |             set_param([gcb '/f32IntegPartK_1FW_Out'], 'Port', '8');
      |             set_param([gcb '/f16InK_1FW_Out'], 'Port', '9');
      |             set_param([gcb '/f32State_Out'], 'Port', '10');
      |         end
      | 
      |         set_param(gcb,'MaskEnables',{'on','on','on','off','off','off','off','off','off','off','off','off','off','off','off','off','off','off','off'});
      | 
      |         if (posblk(4) - posblk(2)) < 875
      |           height = 875;
      |           set_param(gcb,'Position',[posblk(1), posblk(2), posblk(3), posblk(2)+height])
      |         end
      |     else
      |         if (showDebugOutputs == 2) && (strcmp(get_param([gcb '/f16WReqFilt'], 'BlockType'), 'Terminator'))
      |             % shown debugging outputs
      |             pos = get_param(    [gcb '/f16WReqFilt'], 'Position');
      |             orient = get_param( [gcb '/f16WReqFilt'], 'Orientation');
      |             delete_block(       [gcb '/f16WReqFilt']);
      |             add_block('built-in/Outport', [gcb '/f16WReqFilt'], 'Position', pos, 'Orientation', orient);
      | 
      |             pos = get_param(    [gcb '/f16WErr'], 'Position');
      |             orient = get_param( [gcb '/f16WErr'], 'Orientation');
      |             delete_block(       [gcb '/f16WErr']);
      |             add_block('built-in/Outport', [gcb '/f16WErr'], 'Position', pos, 'Orientation', orient);
      | 
      |             pos = get_param(    [gcb '/f16IDQReqAmp'], 'Position');
      |             orient = get_param( [gcb '/f16IDQReqAmp'], 'Orientation');
      |             delete_block(       [gcb '/f16IDQReqAmp']);
      |             add_block('built-in/Outport', [gcb '/f16IDQReqAmp'], 'Position', pos, 'Orientation', orient);
      | 
      |             pos = get_param(    [gcb '/f16WFbckFilt'], 'Position');
      |             orient = get_param( [gcb '/f16WFbckFilt'], 'Orientation');
      |             delete_block(       [gcb '/f16WFbckFilt']);
      |             add_block('built-in/Outport', [gcb '/f16WFbckFilt'], 'Position', pos, 'Orientation', orient);
      | 
      |             pos = get_param(    [gcb '/f16IQErrSign'], 'Position');
      |             orient = get_param( [gcb '/f16IQErrSign'], 'Orientation');
      |             delete_block(       [gcb '/f16IQErrSign']);
      |             add_block('built-in/Outport', [gcb '/f16IQErrSign'], 'Position', pos, 'Orientation', orient);
      | 
      |             pos = get_param(    [gcb '/f16IQErr'], 'Position');
      |             orient = get_param( [gcb '/f16IQErr'], 'Orientation');
      |             delete_block(       [gcb '/f16IQErr']);
      |             add_block('built-in/Outport', [gcb '/f16IQErr'], 'Position', pos, 'Orientation', orient);
      | 
      |             pos = get_param(    [gcb '/f16FWErr'], 'Position');
      |             orient = get_param( [gcb '/f16FWErr'], 'Orientation');
      |             delete_block(       [gcb '/f16FWErr']);
      |             add_block('built-in/Outport', [gcb '/f16FWErr'], 'Position', pos, 'Orientation', orient);
      | 
      |             pos = get_param(    [gcb '/f16UQErr'], 'Position');
      |             orient = get_param( [gcb '/f16UQErr'], 'Orientation');
      |             delete_block(       [gcb '/f16UQErr']);
      |             add_block('built-in/Outport', [gcb '/f16UQErr'], 'Position', pos, 'Orientation', orient);
      | 
      |             pos = get_param(    [gcb '/f16FWErrFilt'], 'Position');
      |             orient = get_param( [gcb '/f16FWErrFilt'], 'Orientation');
      |             delete_block(       [gcb '/f16FWErrFilt']);
      |             add_block('built-in/Outport', [gcb '/f16FWErrFilt'], 'Position', pos, 'Orientation', orient);
      | 
      |             pos = get_param(    [gcb '/f16FWAngle'], 'Position');
      |             orient = get_param( [gcb '/f16FWAngle'], 'Orientation');
      |             delete_block(       [gcb '/f16FWAngle']);
      |             add_block('built-in/Outport', [gcb '/f16FWAngle'], 'Position', pos, 'Orientation', orient);
      | 
      |             pos = get_param(    [gcb '/f16FWSin'], 'Position');
      |             orient = get_param( [gcb '/f16FWSin'], 'Orientation');
      |             delete_block(       [gcb '/f16FWSin']);
      |             add_block('built-in/Outport', [gcb '/f16FWSin'], 'Position', pos, 'Orientation', orient);
      | 
      |             pos = get_param(    [gcb '/f16FWCos'], 'Position');
      |             orient = get_param( [gcb '/f16FWCos'], 'Orientation');
      |             delete_block(       [gcb '/f16FWCos']);
      |             add_block('built-in/Outport', [gcb '/f16FWCos'], 'Position', pos, 'Orientation', orient);
      | 
      |             set_param([gcb '/pIDQReq'], 'Port', '1');
      |             set_param([gcb '/u16LimitFlagQ'], 'Port', '2');
      |             set_param([gcb '/u16LimitFlagFW'], 'Port', '3');
      |             set_param([gcb '/f16WReqFilt'], 'Port', '4');
      |             set_param([gcb '/f16WErr'], 'Port', '5');
      |             set_param([gcb '/f16IDQReqAmp'], 'Port', '6');
      |             set_param([gcb '/f16WFbckFilt'], 'Port', '7');
      |             set_param([gcb '/f16IQErrSign'], 'Port', '8');
      |             set_param([gcb '/f16IQErr'], 'Port', '9');
      |             set_param([gcb '/f16FWErr'], 'Port', '10');
      |             set_param([gcb '/f16UQErr'], 'Port', '11');
      |             set_param([gcb '/f16FWErrFilt'], 'Port', '12');
      |             set_param([gcb '/f16FWAngle'], 'Port', '13');
      |             set_param([gcb '/f16FWSin'], 'Port', '14');
      |             set_param([gcb '/f16FWCos'], 'Port', '15');
      |             set_param([gcb '/f32AccW_Out'], 'Port', '16');
      |             set_param([gcb '/f32AccFW_Out'], 'Port', '17');
      |             set_param([gcb '/f32IntegPartK_1Q_Out'], 'Port', '18');
      |             set_param([gcb '/f16InK_1Q_Out'], 'Port', '19');
      |             set_param([gcb '/f32IntegPartK_1FW_Out'], 'Port', '20');
      |             set_param([gcb '/f16InK_1FW_Out'], 'Port', '21');
      |             set_param([gcb '/f32State_Out'], 'Port', '22');
      |         elseif (showDebugOutputs == 1) && (strcmp(get_param([gcb '/f16WReqFilt'], 'BlockType'), 'Outport'))
      |             % hidden debugging outputs
      |             pos = get_param(    [gcb '/f16WReqFilt'], 'Position');
      |             orient = get_param( [gcb '/f16WReqFilt'], 'Orientation');
      |             delete_block(       [gcb '/f16WReqFilt']);
      |             add_block('built-in/Terminator', [gcb '/f16WReqFilt'], 'Position', pos, 'Orientation', orient);
      | 
      |             pos = get_param(    [gcb '/f16WErr'], 'Position');
      |             orient = get_param( [gcb '/f16WErr'], 'Orientation');
      |             delete_block(       [gcb '/f16WErr']);
      |             add_block('built-in/Terminator', [gcb '/f16WErr'], 'Position', pos, 'Orientation', orient);
      | 
      |             pos = get_param(    [gcb '/f16IDQReqAmp'], 'Position');
      |             orient = get_param( [gcb '/f16IDQReqAmp'], 'Orientation');
      |             delete_block(       [gcb '/f16IDQReqAmp']);
      |             add_block('built-in/Terminator', [gcb '/f16IDQReqAmp'], 'Position', pos, 'Orientation', orient);
      | 
      |             pos = get_param(    [gcb '/f16WFbckFilt'], 'Position');
      |             orient = get_param( [gcb '/f16WFbckFilt'], 'Orientation');
      |             delete_block(       [gcb '/f16WFbckFilt']);
      |             add_block('built-in/Terminator', [gcb '/f16WFbckFilt'], 'Position', pos, 'Orientation', orient);
      | 
      |             pos = get_param(    [gcb '/f16IQErrSign'], 'Position');
      |             orient = get_param( [gcb '/f16IQErrSign'], 'Orientation');
      |             delete_block(       [gcb '/f16IQErrSign']);
      |             add_block('built-in/Terminator', [gcb '/f16IQErrSign'], 'Position', pos, 'Orientation', orient);
      | 
      |             pos = get_param(    [gcb '/f16IQErr'], 'Position');
      |             orient = get_param( [gcb '/f16IQErr'], 'Orientation');
      |             delete_block(       [gcb '/f16IQErr']);
      |             add_block('built-in/Terminator', [gcb '/f16IQErr'], 'Position', pos, 'Orientation', orient);
      | 
      |             pos = get_param(    [gcb '/f16FWErr'], 'Position');
      |             orient = get_param( [gcb '/f16FWErr'], 'Orientation');
      |             delete_block(       [gcb '/f16FWErr']);
      |             add_block('built-in/Terminator', [gcb '/f16FWErr'], 'Position', pos, 'Orientation', orient);
      | 
      |             pos = get_param(    [gcb '/f16UQErr'], 'Position');
      |             orient = get_param( [gcb '/f16UQErr'], 'Orientation');
      |             delete_block(       [gcb '/f16UQErr']);
      |             add_block('built-in/Terminator', [gcb '/f16UQErr'], 'Position', pos, 'Orientation', orient);
      | 
      |             pos = get_param(    [gcb '/f16FWErrFilt'], 'Position');
      |             orient = get_param( [gcb '/f16FWErrFilt'], 'Orientation');
      |             delete_block(       [gcb '/f16FWErrFilt']);
      |             add_block('built-in/Terminator', [gcb '/f16FWErrFilt'], 'Position', pos, 'Orientation', orient);
      | 
      |             pos = get_param(    [gcb '/f16FWAngle'], 'Position');
      |             orient = get_param( [gcb '/f16FWAngle'], 'Orientation');
      |             delete_block(       [gcb '/f16FWAngle']);
      |             add_block('built-in/Terminator', [gcb '/f16FWAngle'], 'Position', pos, 'Orientation', orient);
      | 
      |             pos = get_param(    [gcb '/f16FWSin'], 'Position');
      |             orient = get_param( [gcb '/f16FWSin'], 'Orientation');
      |             delete_block(       [gcb '/f16FWSin']);
      |             add_block('built-in/Terminator', [gcb '/f16FWSin'], 'Position', pos, 'Orientation', orient);
      | 
      |             pos = get_param(    [gcb '/f16FWCos'], 'Position');
      |             orient = get_param( [gcb '/f16FWCos'], 'Orientation');
      |             delete_block(       [gcb '/f16FWCos']);
      |             add_block('built-in/Terminator', [gcb '/f16FWCos'], 'Position', pos, 'Orientation', orient);
      | 
      |             set_param([gcb '/pIDQReq'], 'Port', '1');
      |             set_param([gcb '/u16LimitFlagQ'], 'Port', '2');
      |             set_param([gcb '/u16LimitFlagFW'], 'Port', '3');
      |             set_param([gcb '/f32AccW_Out'], 'Port', '4');
      |             set_param([gcb '/f32AccFW_Out'], 'Port', '5');
      |             set_param([gcb '/f32IntegPartK_1Q_Out'], 'Port', '6');
      |             set_param([gcb '/f16InK_1Q_Out'], 'Port', '7');
      |             set_param([gcb '/f32IntegPartK_1FW_Out'], 'Port', '8');
      |             set_param([gcb '/f16InK_1FW_Out'], 'Port', '9');
      |             set_param([gcb '/f32State_Out'], 'Port', '10');
      |         end
      |     end
      | end
      settings: RTWSystemCode=Inline
      mask TypeOptions showStates: Hide (faster execution) | Show (allows debugging; connect feedback loops manually)
      mask Callback showStates:
      | maskStr = get_param(gcb,'showStates');
      | if strcmp(maskStr,'Hide (faster execution)'),
      |     set_param(gcb,'MaskEnables',{'on','on','off','on','on','on','on','on','on','on','on','on','on','on','on','on','on','on','on'});
      | else
      |     set_param(gcb,'MaskEnables',{'on','on','on','off','off','off','off','off','off','off','off','off','off','off','off','off','off','off','off'});
      | end
      mask TypeOptions resetStatesEnable: Pre-set according to the first set of inputs after reset | Clear to zero
      mask TypeOptions showDebugOutputs: Hide | Show
      mask Display:
      | color('black');
      | pos = get_param(gcb, 'Position');
      | width = pos(3) - pos(1);
      | height = pos(4) - pos(2);
      | tX=width/2;
      | tY=height - 25;
      | color('black');
      | text(tX,tY, 'AMCLIB_FWSpeedLoop_F16', 'horizontalAlignment', 'center');
      | if showStates == 2
      |   color('red');
      |   text(tX,tY - 20, ['debugging mode' char(13) char(10) '(limited performance)'], 'horizontalAlignment', 'center');
      | end
  AMCLIB_FW_F16 : Subsystem  TreatAsAtomicUnit=on  mask(AMCLIB_FW_F16){showStates=Hide (faster execution), resetStatesEnable=Pre-set according to the first set of inputs after reset, showDebugOutputs=Hide, u16NSamples=0, f16PropGain=0, f16IntegGain=0, s16PropGainShift=0, s16IntegGainShift=0, f16LowerLimit=0, f16UpperLimit=0}
      mask prompts: showStates "Show internal states"; resetStatesEnable "Internal state after reset"; showDebugOutputs "Show debugging outputs"; u16NSamples "u16NSamples (GDFLIB_FilterMA - recalculated smoothing factor)"; f16PropGain "f16PropGain (GFLIB_ControllerPIpAW - proportional gain)"; f16IntegGain "f16IntegGain (GFLIB_ControllerPIpAW - integral gain)"; s16PropGainShift "s16PropGainShift (GFLIB_ControllerPIpAW - scaling bitwise shift applied to the proportional gain)"; s16IntegGainShift "s16IntegGainShift (GFLIB_ControllerPIpAW - scaling bitwise shift applied to the integral gain)"; f16LowerLimit "f16LowerLimit (GFLIB_ControllerPIpAW - lower limit)"; f16UpperLimit "f16UpperLimit (GFLIB_ControllerPIpAW - upper limit)"
      mask help: Field Weakening controller for the PMSM field-oriented control algorithm in 16-bit fixed-point fractional implementation. This block supports re-initialization of the internal state during simulation. If the block is reset, the output of the MA filter and PI controller will be aligned with the inputs f16FilterMAFWOut_preset and f16ControllerPIpAWFWOut_preset. Refer to the AMMCLIB User's Guide for further details.
      mask init:
      | if ~evalin('base','exist(''tS8'',''var'')')
      |   if (2 ~= exist('SWLIBS_Typedefs.mat','file'))
      |       error('File SWLIBS_Typedefs.mat is not on the Matlab path. Please add the AMMCLIB "bam" folder in the Matlab Search Path.');
      |   else
      |       evalin('base', 'load(''SWLIBS_Typedefs.mat'')');
      |   end
      | end
      | if showStates == 1
      |     % hidden state variables
      |     if strcmp(get_param([gcb '/u16NSamples'], 'BlockType'), 'Inport')
      |         posblk = get_param(gcb, 'Position');
      | 
      |         pos = get_param(    [gcb, '/u16NSamples'], 'Position');
      |         orient = get_param( [gcb, '/u16NSamples'], 'Orientation');
      |         delete_block(       [gcb, '/u16NSamples']);
      |         add_block('built-in/Ground', [gcb, '/u16NSamples'], 'Position', pos, 'Orientation', orient);
      | 
      |         pos = get_param(    [gcb, '/f16PropGain'], 'Position');
      |         orient = get_param( [gcb, '/f16PropGain'], 'Orientation');
      |         delete_block(       [gcb, '/f16PropGain']);
      |         add_block('built-in/Ground', [gcb, '/f16PropGain'], 'Position', pos, 'Orientation', orient);
      | 
      |         pos = get_param(    [gcb, '/f16IntegGain'], 'Position');
      |         orient = get_param( [gcb, '/f16IntegGain'], 'Orientation');
      |         delete_block(       [gcb, '/f16IntegGain']);
      |         add_block('built-in/Ground', [gcb, '/f16IntegGain'], 'Position', pos, 'Orientation', orient);
      | 
      |         pos = get_param(    [gcb, '/s16PropGainShift'], 'Position');
      |         orient = get_param( [gcb, '/s16PropGainShift'], 'Orientation');
      |         delete_block(       [gcb, '/s16PropGainShift']);
      |         add_block('built-in/Ground', [gcb, '/s16PropGainShift'], 'Position', pos, 'Orientation', orient);
      | 
      |         pos = get_param(    [gcb, '/s16IntegGainShift'], 'Position');
      |         orient = get_param( [gcb, '/s16IntegGainShift'], 'Orientation');
      |         delete_block(       [gcb, '/s16IntegGainShift']);
      |         add_block('built-in/Ground', [gcb, '/s16IntegGainShift'], 'Position', pos, 'Orientation', orient);
      | 
      |         pos = get_param(    [gcb, '/f16LowerLimit'], 'Position');
      |         orient = get_param( [gcb, '/f16LowerLimit'], 'Orientation');
      |         delete_block(       [gcb, '/f16LowerLimit']);
      |         add_block('built-in/Ground', [gcb, '/f16LowerLimit'], 'Position', pos, 'Orientation', orient);
      | 
      |         pos = get_param(    [gcb, '/f16UpperLimit'], 'Position');
      |         orient = get_param( [gcb, '/f16UpperLimit'], 'Orientation');
      |         delete_block(       [gcb, '/f16UpperLimit']);
      |         add_block('built-in/Ground', [gcb, '/f16UpperLimit'], 'Position', pos, 'Orientation', orient);
      | 
      |         pos = get_param(    [gcb, '/f16IQReqK_1'], 'Position');
      |         orient = get_param( [gcb, '/f16IQReqK_1'], 'Orientation');
      |         delete_block(       [gcb, '/f16IQReqK_1']);
      |         add_block('built-in/Ground', [gcb, '/f16IQReqK_1'], 'Position', pos, 'Orientation', orient);
      | 
      |         pos = get_param(    [gcb, '/f32Acc'], 'Position');
      |         orient = get_param( [gcb, '/f32Acc'], 'Orientation');
      |         delete_block(       [gcb, '/f32Acc']);
      |         add_block('built-in/Ground', [gcb, '/f32Acc'], 'Position', pos, 'Orientation', orient);
      | 
      |         pos = get_param(    [gcb, '/f32IntegPartK_1'], 'Position');
      |         orient = get_param( [gcb, '/f32IntegPartK_1'], 'Orientation');
      |         delete_block(       [gcb, '/f32IntegPartK_1']);
      |         add_block('built-in/Ground', [gcb, '/f32IntegPartK_1'], 'Position', pos, 'Orientation', orient);
      | 
      |         pos = get_param(    [gcb, '/f16InK_1'], 'Position');
      |         orient = get_param( [gcb, '/f16InK_1'], 'Orientation');
      |         delete_block(       [gcb, '/f16InK_1']);
      |         add_block('built-in/Ground', [gcb, '/f16InK_1'], 'Position', pos, 'Orientation', orient);
      | 
      | 
      |         pos = get_param(    [gcb '/f32Acc_Out'], 'Position');
      |         orient = get_param( [gcb '/f32Acc_Out'], 'Orientation');
      |         delete_block(       [gcb '/f32Acc_Out']);
      |         add_block('built-in/Terminator', [gcb '/f32Acc_Out'], 'Position', pos, 'Orientation', orient);
      | 
      |         pos = get_param(    [gcb '/f32IntegPartK_1_Out'], 'Position');
      |         orient = get_param( [gcb '/f32IntegPartK_1_Out'], 'Orientation');
      |         delete_block(       [gcb '/f32IntegPartK_1_Out']);
      |         add_block('built-in/Terminator', [gcb '/f32IntegPartK_1_Out'], 'Position', pos, 'Orientation', orient);
      | 
      |         pos = get_param(    [gcb '/f16InK_1_Out'], 'Position');
      |         orient = get_param( [gcb '/f16InK_1_Out'], 'Orientation');
      |         delete_block(       [gcb '/f16InK_1_Out']);
      |         add_block('built-in/Terminator', [gcb '/f16InK_1_Out'], 'Position', pos, 'Orientation', orient);
      | 
      | 
      |         if strcmp(get_param([gcb '/f16IQErrSign'], 'BlockType'), 'Outport')
      |             pos = get_param(    [gcb '/f16IQErrSign'], 'Position');
      |             orient = get_param( [gcb '/f16IQErrSign'], 'Orientation');
      |             delete_block(       [gcb '/f16IQErrSign']);
      |             add_block('built-in/Terminator', [gcb '/f16IQErrSign'], 'Position', pos, 'Orientation', orient);
      | 
      |             pos = get_param(    [gcb '/f16IQErr'], 'Position');
      |             orient = get_param( [gcb '/f16IQErr'], 'Orientation');
      |             delete_block(       [gcb '/f16IQErr']);
      |             add_block('built-in/Terminator', [gcb '/f16IQErr'], 'Position', pos, 'Orientation', orient);
      | 
      |             pos = get_param(    [gcb '/f16FWErr'], 'Position');
      |             orient = get_param( [gcb '/f16FWErr'], 'Orientation');
      |             delete_block(       [gcb '/f16FWErr']);
      |             add_block('built-in/Terminator', [gcb '/f16FWErr'], 'Position', pos, 'Orientation', orient);
      | 
      |             pos = get_param(    [gcb '/f16UQErr'], 'Position');
      |             orient = get_param( [gcb '/f16UQErr'], 'Orientation');
      |             delete_block(       [gcb '/f16UQErr']);
      |             add_block('built-in/Terminator', [gcb '/f16UQErr'], 'Position', pos, 'Orientation', orient);
      | 
      |             pos = get_param(    [gcb '/f16FWErrFilt'], 'Position');
      |             orient = get_param( [gcb '/f16FWErrFilt'], 'Orientation');
      |             delete_block(       [gcb '/f16FWErrFilt']);
      |             add_block('built-in/Terminator', [gcb '/f16FWErrFilt'], 'Position', pos, 'Orientation', orient);
      | 
      |             pos = get_param(    [gcb '/f16FWAngle'], 'Position');
      |             orient = get_param( [gcb '/f16FWAngle'], 'Orientation');
      |             delete_block(       [gcb '/f16FWAngle']);
      |             add_block('built-in/Terminator', [gcb '/f16FWAngle'], 'Position', pos, 'Orientation', orient);
      | 
      |             pos = get_param(    [gcb '/f16FWSin'], 'Position');
      |             orient = get_param( [gcb '/f16FWSin'], 'Orientation');
      |             delete_block(       [gcb '/f16FWSin']);
      |             add_block('built-in/Terminator', [gcb '/f16FWSin'], 'Position', pos, 'Orientation', orient);
      | 
      |             pos = get_param(    [gcb '/f16FWCos'], 'Position');
      |             orient = get_param( [gcb '/f16FWCos'], 'Orientation');
      |             delete_block(       [gcb '/f16FWCos']);
      |             add_block('built-in/Terminator', [gcb '/f16FWCos'], 'Position', pos, 'Orientation', orient);
      | 
      |         end
      | 
      |         set_param([gcb '/f16IDQReqAmp'], 'Port', '1');
      |         set_param([gcb '/f16VelocityFbck'], 'Port', '2');
      |         set_param([gcb '/f16IQFbck'], 'Port', '3');
      |         set_param([gcb '/f16UQReq'], 'Port', '4');
      |         set_param([gcb '/f16UQLim'], 'Port', '5');
      |         set_param([gcb '/f16FilterMAFWOut_preset'], 'Port', '6');
      |         set_param([gcb '/f16ControllerPIpAWFWOut_preset'], 'Port', '7');
      | 
      |         set_param([gcb '/pIDQReq'], 'Port', '1');
      |         set_param([gcb '/u16LimitFlag'], 'Port', '2');
      | 
      |         set_param(gcb,'MaskEnables',{'on','on','off','on','on','on','on','on','on','on'});
      | 
      |         if (posblk(4) - posblk(2)) > 200
      |           height = 200;
      |           set_param(gcb,'Position',[posblk(1), posblk(2), posblk(3), posblk(2)+height])
      |         end
      |     end
      | else
      |     % shown state variables
      |     if strcmp(get_param([gcb '/u16NSamples'], 'BlockType'), 'Ground')
      |         posblk = get_param(gcb, 'Position');
      | 
      |         pos = get_param(    [gcb, '/u16NSamples'], 'Position');
      |         orient = get_param( [gcb, '/u16NSamples'], 'Orientation');
      |         delete_block(       [gcb, '/u16NSamples']);
      |         add_block('built-in/Inport', [gcb, '/u16NSamples'], 'Position', pos, 'Orientation', orient, 'OutDataTypeStr', 'uint16');
      | 
      |         pos = get_param(    [gcb, '/f16PropGain'], 'Position');
      |         orient = get_param( [gcb, '/f16PropGain'], 'Orientation');
      |         delete_block(       [gcb, '/f16PropGain']);
      |         add_block('built-in/Inport', [gcb, '/f16PropGain'], 'Position', pos, 'Orientation', orient, 'OutDataTypeStr', 'int16');
      | 
      |         pos = get_param(    [gcb, '/f16IntegGain'], 'Position');
      |         orient = get_param( [gcb, '/f16IntegGain'], 'Orientation');
      |         delete_block(       [gcb, '/f16IntegGain']);
      |         add_block('built-in/Inport', [gcb, '/f16IntegGain'], 'Position', pos, 'Orientation', orient, 'OutDataTypeStr', 'int16');
      | 
      |         pos = get_param(    [gcb, '/s16PropGainShift'], 'Position');
      |         orient = get_param( [gcb, '/s16PropGainShift'], 'Orientation');
      |         delete_block(       [gcb, '/s16PropGainShift']);
      |         add_block('built-in/Inport', [gcb, '/s16PropGainShift'], 'Position', pos, 'Orientation', orient, 'OutDataTypeStr', 'int16');
      | 
      |         pos = get_param(    [gcb, '/s16IntegGainShift'], 'Position');
      |         orient = get_param( [gcb, '/s16IntegGainShift'], 'Orientation');
      |         delete_block(       [gcb, '/s16IntegGainShift']);
      |         add_block('built-in/Inport', [gcb, '/s16IntegGainShift'], 'Position', pos, 'Orientation', orient, 'OutDataTypeStr', 'int16');
      | 
      |         pos = get_param(    [gcb, '/f16LowerLimit'], 'Position');
      |         orient = get_param( [gcb, '/f16LowerLimit'], 'Orientation');
      |         delete_block(       [gcb, '/f16LowerLimit']);
      |         add_block('built-in/Inport', [gcb, '/f16LowerLimit'], 'Position', pos, 'Orientation', orient, 'OutDataTypeStr', 'int16');
      | 
      |         pos = get_param(    [gcb, '/f16UpperLimit'], 'Position');
      |         orient = get_param( [gcb, '/f16UpperLimit'], 'Orientation');
      |         delete_block(       [gcb, '/f16UpperLimit']);
      |         add_block('built-in/Inport', [gcb, '/f16UpperLimit'], 'Position', pos, 'Orientation', orient, 'OutDataTypeStr', 'int16');
      | 
      |         pos = get_param(    [gcb, '/f16IQReqK_1'], 'Position');
      |         orient = get_param( [gcb, '/f16IQReqK_1'], 'Orientation');
      |         delete_block(       [gcb, '/f16IQReqK_1']);
      |         add_block('built-in/Inport', [gcb, '/f16IQReqK_1'], 'Position', pos, 'Orientation', orient, 'OutDataTypeStr', 'int16');
      | 
      |         pos = get_param(    [gcb, '/f32Acc'], 'Position');
      |         orient = get_param( [gcb, '/f32Acc'], 'Orientation');
      |         delete_block(       [gcb, '/f32Acc']);
      |         add_block('built-in/Inport', [gcb, '/f32Acc'], 'Position', pos, 'Orientation', orient, 'OutDataTypeStr', 'int32');
      | 
      |         pos = get_param(    [gcb, '/f32IntegPartK_1'], 'Position');
      |         orient = get_param( [gcb, '/f32IntegPartK_1'], 'Orientation');
      |         delete_block(       [gcb, '/f32IntegPartK_1']);
      |         add_block('built-in/Inport', [gcb, '/f32IntegPartK_1'], 'Position', pos, 'Orientation', orient, 'OutDataTypeStr', 'int32');
      | 
      |         pos = get_param(    [gcb, '/f16InK_1'], 'Position');
      |         orient = get_param( [gcb, '/f16InK_1'], 'Orientation');
      |         delete_block(       [gcb, '/f16InK_1']);
      |         add_block('built-in/Inport', [gcb, '/f16InK_1'], 'Position', pos, 'Orientation', orient, 'OutDataTypeStr', 'int16');
      | 
      | 
      |         pos = get_param(    [gcb '/f32Acc_Out'], 'Position');
      |         orient = get_param( [gcb '/f32Acc_Out'], 'Orientation');
      |         delete_block(       [gcb '/f32Acc_Out']);
      |         add_block('built-in/Outport', [gcb '/f32Acc_Out'], 'Position', pos, 'Orientation', orient);
      | 
      |         pos = get_param(    [gcb '/f32IntegPartK_1_Out'], 'Position');
      |         orient = get_param( [gcb '/f32IntegPartK_1_Out'], 'Orientation');
      |         delete_block(       [gcb '/f32IntegPartK_1_Out']);
      |         add_block('built-in/Outport', [gcb '/f32IntegPartK_1_Out'], 'Position', pos, 'Orientation', orient);
      | 
      |         pos = get_param(    [gcb '/f16InK_1_Out'], 'Position');
      |         orient = get_param( [gcb '/f16InK_1_Out'], 'Orientation');
      |         delete_block(       [gcb '/f16InK_1_Out']);
      |         add_block('built-in/Outport', [gcb '/f16InK_1_Out'], 'Position', pos, 'Orientation', orient);
      | 
      | 
      |         if (showDebugOutputs == 2) && (strcmp(get_param([gcb '/f16IQErrSign'], 'BlockType'), 'Terminator'))
      |             pos = get_param(    [gcb '/f16IQErrSign'], 'Position');
      |             orient = get_param( [gcb '/f16IQErrSign'], 'Orientation');
      |             delete_block(       [gcb '/f16IQErrSign']);
      |             add_block('built-in/Outport', [gcb '/f16IQErrSign'], 'Position', pos, 'Orientation', orient);
      | 
      |             pos = get_param(    [gcb '/f16IQErr'], 'Position');
      |             orient = get_param( [gcb '/f16IQErr'], 'Orientation');
      |             delete_block(       [gcb '/f16IQErr']);
      |             add_block('built-in/Outport', [gcb '/f16IQErr'], 'Position', pos, 'Orientation', orient);
      | 
      |             pos = get_param(    [gcb '/f16FWErr'], 'Position');
      |             orient = get_param( [gcb '/f16FWErr'], 'Orientation');
      |             delete_block(       [gcb '/f16FWErr']);
      |             add_block('built-in/Outport', [gcb '/f16FWErr'], 'Position', pos, 'Orientation', orient);
      | 
      |             pos = get_param(    [gcb '/f16UQErr'], 'Position');
      |             orient = get_param( [gcb '/f16UQErr'], 'Orientation');
      |             delete_block(       [gcb '/f16UQErr']);
      |             add_block('built-in/Outport', [gcb '/f16UQErr'], 'Position', pos, 'Orientation', orient);
      | 
      |             pos = get_param(    [gcb '/f16FWErrFilt'], 'Position');
      |             orient = get_param( [gcb '/f16FWErrFilt'], 'Orientation');
      |             delete_block(       [gcb '/f16FWErrFilt']);
      |             add_block('built-in/Outport', [gcb '/f16FWErrFilt'], 'Position', pos, 'Orientation', orient);
      | 
      |             pos = get_param(    [gcb '/f16FWAngle'], 'Position');
      |             orient = get_param( [gcb '/f16FWAngle'], 'Orientation');
      |             delete_block(       [gcb '/f16FWAngle']);
      |             add_block('built-in/Outport', [gcb '/f16FWAngle'], 'Position', pos, 'Orientation', orient);
      | 
      |             pos = get_param(    [gcb '/f16FWSin'], 'Position');
      |             orient = get_param( [gcb '/f16FWSin'], 'Orientation');
      |             delete_block(       [gcb '/f16FWSin']);
      |             add_block('built-in/Outport', [gcb '/f16FWSin'], 'Position', pos, 'Orientation', orient);
      | 
      |             pos = get_param(    [gcb '/f16FWCos'], 'Position');
      |             orient = get_param( [gcb '/f16FWCos'], 'Orientation');
      |             delete_block(       [gcb '/f16FWCos']);
      |             add_block('built-in/Outport', [gcb '/f16FWCos'], 'Position', pos, 'Orientation', orient);
      | 
      |         end
      | 
      |         set_param([gcb '/f16IDQReqAmp'], 'Port', '1');
      |         set_param([gcb '/f16VelocityFbck'], 'Port', '2');
      |         set_param([gcb '/f16IQFbck'], 'Port', '3');
      |         set_param([gcb '/f16UQReq'], 'Port', '4');
      |         set_param([gcb '/f16UQLim'], 'Port', '5');
      |         set_param([gcb '/f16FilterMAFWOut_preset'], 'Port', '6');
      |         set_param([gcb '/f16ControllerPIpAWFWOut_preset'], 'Port', '7');
      |         set_param([gcb '/u16NSamples'], 'Port', '8');
      |         set_param([gcb '/f16PropGain'], 'Port', '9');
      |         set_param([gcb '/f16IntegGain'], 'Port', '10');
      |         set_param([gcb '/s16PropGainShift'], 'Port', '11');
      |         set_param([gcb '/s16IntegGainShift'], 'Port', '12');
      |         set_param([gcb '/f16LowerLimit'], 'Port', '13');
      |         set_param([gcb '/f16UpperLimit'], 'Port', '14');
      |         set_param([gcb '/f16IQReqK_1'], 'Port', '15');
      |         set_param([gcb '/f32Acc'], 'Port', '16');
      |         set_param([gcb '/f32IntegPartK_1'], 'Port', '17');
      |         set_param([gcb '/f16InK_1'], 'Port', '18');
      | 
      |         if (showDebugOutputs == 2)
      |             set_param([gcb '/pIDQReq'], 'Port', '1');
      |             set_param([gcb '/u16LimitFlag'], 'Port', '2');
      |             set_param([gcb '/f16IQErrSign'], 'Port', '3');
      |             set_param([gcb '/f16IQErr'], 'Port', '4');
      |             set_param([gcb '/f16FWErr'], 'Port', '5');
      |             set_param([gcb '/f16UQErr'], 'Port', '6');
      |             set_param([gcb '/f16FWErrFilt'], 'Port', '7');
      |             set_param([gcb '/f16FWAngle'], 'Port', '8');
      |             set_param([gcb '/f16FWSin'], 'Port', '9');
      |             set_param([gcb '/f16FWCos'], 'Port', '10');
      |             set_param([gcb '/f32Acc_Out'], 'Port', '11');
      |             set_param([gcb '/f32IntegPartK_1_Out'], 'Port', '12');
      |             set_param([gcb '/f16InK_1_Out'], 'Port', '13');
      |         else
      |             set_param([gcb '/pIDQReq'], 'Port', '1');
      |             set_param([gcb '/u16LimitFlag'], 'Port', '2');
      |             set_param([gcb '/f32Acc_Out'], 'Port', '3');
      |             set_param([gcb '/f32IntegPartK_1_Out'], 'Port', '4');
      |             set_param([gcb '/f16InK_1_Out'], 'Port', '5');
      |         end
      | 
      |         set_param(gcb,'MaskEnables',{'on','on','on','off','off','off','off','off','off','off'});
      | 
      |         if (posblk(4) - posblk(2)) < 475
      |           height = 475;
      |           set_param(gcb,'Position',[posblk(1), posblk(2), posblk(3), posblk(2)+height])
      |         end
      |     else
      |         if (showDebugOutputs == 2) && (strcmp(get_param([gcb '/f16IQErrSign'], 'BlockType'), 'Terminator'))
      |             % shown debugging outputs
      |             pos = get_param(    [gcb '/f16IQErrSign'], 'Position');
      |             orient = get_param( [gcb '/f16IQErrSign'], 'Orientation');
      |             delete_block(       [gcb '/f16IQErrSign']);
      |             add_block('built-in/Outport', [gcb '/f16IQErrSign'], 'Position', pos, 'Orientation', orient);
      | 
      |             pos = get_param(    [gcb '/f16IQErr'], 'Position');
      |             orient = get_param( [gcb '/f16IQErr'], 'Orientation');
      |             delete_block(       [gcb '/f16IQErr']);
      |             add_block('built-in/Outport', [gcb '/f16IQErr'], 'Position', pos, 'Orientation', orient);
      | 
      |             pos = get_param(    [gcb '/f16FWErr'], 'Position');
      |             orient = get_param( [gcb '/f16FWErr'], 'Orientation');
      |             delete_block(       [gcb '/f16FWErr']);
      |             add_block('built-in/Outport', [gcb '/f16FWErr'], 'Position', pos, 'Orientation', orient);
      | 
      |             pos = get_param(    [gcb '/f16UQErr'], 'Position');
      |             orient = get_param( [gcb '/f16UQErr'], 'Orientation');
      |             delete_block(       [gcb '/f16UQErr']);
      |             add_block('built-in/Outport', [gcb '/f16UQErr'], 'Position', pos, 'Orientation', orient);
      | 
      |             pos = get_param(    [gcb '/f16FWErrFilt'], 'Position');
      |             orient = get_param( [gcb '/f16FWErrFilt'], 'Orientation');
      |             delete_block(       [gcb '/f16FWErrFilt']);
      |             add_block('built-in/Outport', [gcb '/f16FWErrFilt'], 'Position', pos, 'Orientation', orient);
      | 
      |             pos = get_param(    [gcb '/f16FWAngle'], 'Position');
      |             orient = get_param( [gcb '/f16FWAngle'], 'Orientation');
      |             delete_block(       [gcb '/f16FWAngle']);
      |             add_block('built-in/Outport', [gcb '/f16FWAngle'], 'Position', pos, 'Orientation', orient);
      | 
      |             pos = get_param(    [gcb '/f16FWSin'], 'Position');
      |             orient = get_param( [gcb '/f16FWSin'], 'Orientation');
      |             delete_block(       [gcb '/f16FWSin']);
      |             add_block('built-in/Outport', [gcb '/f16FWSin'], 'Position', pos, 'Orientation', orient);
      | 
      |             pos = get_param(    [gcb '/f16FWCos'], 'Position');
      |             orient = get_param( [gcb '/f16FWCos'], 'Orientation');
      |             delete_block(       [gcb '/f16FWCos']);
      |             add_block('built-in/Outport', [gcb '/f16FWCos'], 'Position', pos, 'Orientation', orient);
      | 
      |             set_param([gcb '/pIDQReq'], 'Port', '1');
      |             set_param([gcb '/u16LimitFlag'], 'Port', '2');
      |             set_param([gcb '/f16IQErrSign'], 'Port', '3');
      |             set_param([gcb '/f16IQErr'], 'Port', '4');
      |             set_param([gcb '/f16FWErr'], 'Port', '5');
      |             set_param([gcb '/f16UQErr'], 'Port', '6');
      |             set_param([gcb '/f16FWErrFilt'], 'Port', '7');
      |             set_param([gcb '/f16FWAngle'], 'Port', '8');
      |             set_param([gcb '/f16FWSin'], 'Port', '9');
      |             set_param([gcb '/f16FWCos'], 'Port', '10');
      |             set_param([gcb '/f32Acc_Out'], 'Port', '11');
      |             set_param([gcb '/f32IntegPartK_1_Out'], 'Port', '12');
      |             set_param([gcb '/f16InK_1_Out'], 'Port', '13');
      |         elseif (showDebugOutputs == 1) && (strcmp(get_param([gcb '/f16IQErrSign'], 'BlockType'), 'Outport'))
      |             % hidden debugging outputs
      |             pos = get_param(    [gcb '/f16IQErrSign'], 'Position');
      |             orient = get_param( [gcb '/f16IQErrSign'], 'Orientation');
      |             delete_block(       [gcb '/f16IQErrSign']);
      |             add_block('built-in/Terminator', [gcb '/f16IQErrSign'], 'Position', pos, 'Orientation', orient);
      | 
      |             pos = get_param(    [gcb '/f16IQErr'], 'Position');
      |             orient = get_param( [gcb '/f16IQErr'], 'Orientation');
      |             delete_block(       [gcb '/f16IQErr']);
      |             add_block('built-in/Terminator', [gcb '/f16IQErr'], 'Position', pos, 'Orientation', orient);
      | 
      |             pos = get_param(    [gcb '/f16FWErr'], 'Position');
      |             orient = get_param( [gcb '/f16FWErr'], 'Orientation');
      |             delete_block(       [gcb '/f16FWErr']);
      |             add_block('built-in/Terminator', [gcb '/f16FWErr'], 'Position', pos, 'Orientation', orient);
      | 
      |             pos = get_param(    [gcb '/f16UQErr'], 'Position');
      |             orient = get_param( [gcb '/f16UQErr'], 'Orientation');
      |             delete_block(       [gcb '/f16UQErr']);
      |             add_block('built-in/Terminator', [gcb '/f16UQErr'], 'Position', pos, 'Orientation', orient);
      | 
      |             pos = get_param(    [gcb '/f16FWErrFilt'], 'Position');
      |             orient = get_param( [gcb '/f16FWErrFilt'], 'Orientation');
      |             delete_block(       [gcb '/f16FWErrFilt']);
      |             add_block('built-in/Terminator', [gcb '/f16FWErrFilt'], 'Position', pos, 'Orientation', orient);
      | 
      |             pos = get_param(    [gcb '/f16FWAngle'], 'Position');
      |             orient = get_param( [gcb '/f16FWAngle'], 'Orientation');
      |             delete_block(       [gcb '/f16FWAngle']);
      |             add_block('built-in/Terminator', [gcb '/f16FWAngle'], 'Position', pos, 'Orientation', orient);
      | 
      |             pos = get_param(    [gcb '/f16FWSin'], 'Position');
      |             orient = get_param( [gcb '/f16FWSin'], 'Orientation');
      |             delete_block(       [gcb '/f16FWSin']);
      |             add_block('built-in/Terminator', [gcb '/f16FWSin'], 'Position', pos, 'Orientation', orient);
      | 
      |             pos = get_param(    [gcb '/f16FWCos'], 'Position');
      |             orient = get_param( [gcb '/f16FWCos'], 'Orientation');
      |             delete_block(       [gcb '/f16FWCos']);
      |             add_block('built-in/Terminator', [gcb '/f16FWCos'], 'Position', pos, 'Orientation', orient);
      | 
      |             set_param([gcb '/pIDQReq'], 'Port', '1');
      |             set_param([gcb '/u16LimitFlag'], 'Port', '2');
      |             set_param([gcb '/f32Acc_Out'], 'Port', '3');
      |             set_param([gcb '/f32IntegPartK_1_Out'], 'Port', '4');
      |             set_param([gcb '/f16InK_1_Out'], 'Port', '5');
      |         end
      |     end
      | end
      settings: RTWSystemCode=Inline
      mask TypeOptions showStates: Hide (faster execution) | Show (allows debugging; connect feedback loops manually)
      mask Callback showStates:
      | maskStr = get_param(gcb,'showStates');
      | if strcmp(maskStr,'Hide (faster execution)'),
      |     set_param(gcb,'MaskEnables',{'on','on','off','on','on','on','on','on','on','on'});
      | else
      |     set_param(gcb,'MaskEnables',{'on','on','on','off','off','off','off','off','off','off'});
      | end
      mask TypeOptions resetStatesEnable: Pre-set according to the first set of inputs after reset | Clear to zero
      mask TypeOptions showDebugOutputs: Hide | Show
      mask Display:
      | color('black');
      | pos = get_param(gcb, 'Position');
      | width = pos(3) - pos(1);
      | height = pos(4) - pos(2);
      | tX=width/2;
      | tY=height - 25;
      | color('black');
      | text(tX,tY, 'AMCLIB_FW_F16', 'horizontalAlignment', 'center');
      | if showStates == 2
      |   color('red');
      |   text(tX,tY - 20, ['debugging mode' char(13) char(10) '(limited performance)'], 'horizontalAlignment', 'center');
      | end
  AMCLIB_SpeedLoop_F16 : Subsystem  TreatAsAtomicUnit=on  mask(AMCLIB_SpeedLoop_F16){showStates=Hide (faster execution), resetStatesEnable=Pre-set according to the first set of inputs after reset, showDebugOutputs=Hide, u16NSamplesW=0, f16PropGainQ=0, f16IntegGainQ=0, s16PropGainShiftQ=0, s16IntegGainShiftQ=0, f16LowerLimitQ=0, f16UpperLimitQ=0, f32RampUp=0, f32RampDown=0}
      mask prompts: showStates "Show internal states"; resetStatesEnable "Internal state after reset"; showDebugOutputs "Show debugging outputs"; u16NSamplesW "u16NSamplesW (GDFLIB_FilterMA - recalculated smoothing factor)"; f16PropGainQ "f16PropGainQ (GFLIB_ControllerPIpAW - proportional gain)"; f16IntegGainQ "f16IntegGainQ (GFLIB_ControllerPIpAW - integral gain)"; s16PropGainShiftQ "s16PropGainShiftQ (GFLIB_ControllerPIpAW - scaling bitwise shift applied to the proportional gain)"; s16IntegGainShiftQ "s16IntegGainShiftQ (GFLIB_ControllerPIpAW - scaling bitwise shift applied to the integral gain)"; f16LowerLimitQ "f16LowerLimitQ (GFLIB_ControllerPIpAW - lower limit)"; f16UpperLimitQ "f16UpperLimitQ (GFLIB_ControllerPIpAW - upper limit)"; f32RampUp "f32RampUp (Ramp up increment coefficient)"; f32RampDown "f32RampDown (Ramp decrement coefficient)"
      mask help: Speed loop controller for the PMSM field-oriented control algorithm in 16-bit fixed-point fractional implementation. This block supports re-initialization of the internal state during simulation. If the block is reset, the outputs of the MA filter, PI controller, and the ramp will be aligned with the inputs f16FilterMAWOut_preset, f16ControllerPIpAWQOut_preset, and f32RampOut_preset. Refer to the AMMCLIB User's Guide for further details.
      mask init:
      | if ~evalin('base','exist(''tS8'',''var'')')
      |   if (2 ~= exist('SWLIBS_Typedefs.mat','file'))
      |       error('File SWLIBS_Typedefs.mat is not on the Matlab path. Please add the AMMCLIB "bam" folder in the Matlab Search Path.');
      |   else
      |       evalin('base', 'load(''SWLIBS_Typedefs.mat'')');
      |   end
      | end
      | if showStates == 1
      |     % hidden state variables
      |     if strcmp(get_param([gcb '/u16NSamplesW'], 'BlockType'), 'Inport')
      |         posblk = get_param(gcb, 'Position');
      | 
      |         pos = get_param(    [gcb, '/u16NSamplesW'], 'Position');
      |         orient = get_param( [gcb, '/u16NSamplesW'], 'Orientation');
      |         delete_block(       [gcb, '/u16NSamplesW']);
      |         add_block('built-in/Ground', [gcb, '/u16NSamplesW'], 'Position', pos, 'Orientation', orient);
      | 
      |         pos = get_param(    [gcb, '/f16PropGainQ'], 'Position');
      |         orient = get_param( [gcb, '/f16PropGainQ'], 'Orientation');
      |         delete_block(       [gcb, '/f16PropGainQ']);
      |         add_block('built-in/Ground', [gcb, '/f16PropGainQ'], 'Position', pos, 'Orientation', orient);
      | 
      |         pos = get_param(    [gcb, '/f16IntegGainQ'], 'Position');
      |         orient = get_param( [gcb, '/f16IntegGainQ'], 'Orientation');
      |         delete_block(       [gcb, '/f16IntegGainQ']);
      |         add_block('built-in/Ground', [gcb, '/f16IntegGainQ'], 'Position', pos, 'Orientation', orient);
      | 
      |         pos = get_param(    [gcb, '/s16PropGainShiftQ'], 'Position');
      |         orient = get_param( [gcb, '/s16PropGainShiftQ'], 'Orientation');
      |         delete_block(       [gcb, '/s16PropGainShiftQ']);
      |         add_block('built-in/Ground', [gcb, '/s16PropGainShiftQ'], 'Position', pos, 'Orientation', orient);
      | 
      |         pos = get_param(    [gcb, '/s16IntegGainShiftQ'], 'Position');
      |         orient = get_param( [gcb, '/s16IntegGainShiftQ'], 'Orientation');
      |         delete_block(       [gcb, '/s16IntegGainShiftQ']);
      |         add_block('built-in/Ground', [gcb, '/s16IntegGainShiftQ'], 'Position', pos, 'Orientation', orient);
      | 
      |         pos = get_param(    [gcb, '/f16LowerLimitQ'], 'Position');
      |         orient = get_param( [gcb, '/f16LowerLimitQ'], 'Orientation');
      |         delete_block(       [gcb, '/f16LowerLimitQ']);
      |         add_block('built-in/Ground', [gcb, '/f16LowerLimitQ'], 'Position', pos, 'Orientation', orient);
      | 
      |         pos = get_param(    [gcb, '/f16UpperLimitQ'], 'Position');
      |         orient = get_param( [gcb, '/f16UpperLimitQ'], 'Orientation');
      |         delete_block(       [gcb, '/f16UpperLimitQ']);
      |         add_block('built-in/Ground', [gcb, '/f16UpperLimitQ'], 'Position', pos, 'Orientation', orient);
      | 
      |         pos = get_param(    [gcb, '/f32RampUp'], 'Position');
      |         orient = get_param( [gcb, '/f32RampUp'], 'Orientation');
      |         delete_block(       [gcb, '/f32RampUp']);
      |         add_block('built-in/Ground', [gcb, '/f32RampUp'], 'Position', pos, 'Orientation', orient);
      | 
      |         pos = get_param(    [gcb, '/f32RampDown'], 'Position');
      |         orient = get_param( [gcb, '/f32RampDown'], 'Orientation');
      |         delete_block(       [gcb, '/f32RampDown']);
      |         add_block('built-in/Ground', [gcb, '/f32RampDown'], 'Position', pos, 'Orientation', orient);
      | 
      |         pos = get_param(    [gcb, '/f32AccW'], 'Position');
      |         orient = get_param( [gcb, '/f32AccW'], 'Orientation');
      |         delete_block(       [gcb, '/f32AccW']);
      |         add_block('built-in/Ground', [gcb, '/f32AccW'], 'Position', pos, 'Orientation', orient);
      | 
      |         pos = get_param(    [gcb, '/f32IntegPartK_1Q'], 'Position');
      |         orient = get_param( [gcb, '/f32IntegPartK_1Q'], 'Orientation');
      |         delete_block(       [gcb, '/f32IntegPartK_1Q']);
      |         add_block('built-in/Ground', [gcb, '/f32IntegPartK_1Q'], 'Position', pos, 'Orientation', orient);
      | 
      |         pos = get_param(    [gcb, '/f16InK_1Q'], 'Position');
      |         orient = get_param( [gcb, '/f16InK_1Q'], 'Orientation');
      |         delete_block(       [gcb, '/f16InK_1Q']);
      |         add_block('built-in/Ground', [gcb, '/f16InK_1Q'], 'Position', pos, 'Orientation', orient);
      | 
      |         pos = get_param(    [gcb, '/f32State'], 'Position');
      |         orient = get_param( [gcb, '/f32State'], 'Orientation');
      |         delete_block(       [gcb, '/f32State']);
      |         add_block('built-in/Ground', [gcb, '/f32State'], 'Position', pos, 'Orientation', orient);
      | 
      | 
      |         pos = get_param(    [gcb '/f32AccW_Out'], 'Position');
      |         orient = get_param( [gcb '/f32AccW_Out'], 'Orientation');
      |         delete_block(       [gcb '/f32AccW_Out']);
      |         add_block('built-in/Terminator', [gcb '/f32AccW_Out'], 'Position', pos, 'Orientation', orient);
      | 
      |         pos = get_param(    [gcb '/f32IntegPartK_1Q_Out'], 'Position');
      |         orient = get_param( [gcb '/f32IntegPartK_1Q_Out'], 'Orientation');
      |         delete_block(       [gcb '/f32IntegPartK_1Q_Out']);
      |         add_block('built-in/Terminator', [gcb '/f32IntegPartK_1Q_Out'], 'Position', pos, 'Orientation', orient);
      | 
      |         pos = get_param(    [gcb '/f16InK_1Q_Out'], 'Position');
      |         orient = get_param( [gcb '/f16InK_1Q_Out'], 'Orientation');
      |         delete_block(       [gcb '/f16InK_1Q_Out']);
      |         add_block('built-in/Terminator', [gcb '/f16InK_1Q_Out'], 'Position', pos, 'Orientation', orient);
      | 
      |         pos = get_param(    [gcb '/f32State_Out'], 'Position');
      |         orient = get_param( [gcb '/f32State_Out'], 'Orientation');
      |         delete_block(       [gcb '/f32State_Out']);
      |         add_block('built-in/Terminator', [gcb '/f32State_Out'], 'Position', pos, 'Orientation', orient);
      | 
      | 
      |         if strcmp(get_param([gcb '/f16WReqFilt'], 'BlockType'), 'Outport')
      |             pos = get_param(    [gcb '/f16WReqFilt'], 'Position');
      |             orient = get_param( [gcb '/f16WReqFilt'], 'Orientation');
      |             delete_block(       [gcb '/f16WReqFilt']);
      |             add_block('built-in/Terminator', [gcb '/f16WReqFilt'], 'Position', pos, 'Orientation', orient);
      | 
      |             pos = get_param(    [gcb '/f16WErr'], 'Position');
      |             orient = get_param( [gcb '/f16WErr'], 'Orientation');
      |             delete_block(       [gcb '/f16WErr']);
      |             add_block('built-in/Terminator', [gcb '/f16WErr'], 'Position', pos, 'Orientation', orient);
      | 
      |             pos = get_param(    [gcb '/f16WFbckFilt'], 'Position');
      |             orient = get_param( [gcb '/f16WFbckFilt'], 'Orientation');
      |             delete_block(       [gcb '/f16WFbckFilt']);
      |             add_block('built-in/Terminator', [gcb '/f16WFbckFilt'], 'Position', pos, 'Orientation', orient);
      | 
      |         end
      | 
      |         set_param([gcb '/f16VelocityReq'], 'Port', '1');
      |         set_param([gcb '/f16VelocityFbck'], 'Port', '2');
      |         set_param([gcb '/f16FilterMAWOut_preset'], 'Port', '3');
      |         set_param([gcb '/f16ControllerPIpAWQOut_preset'], 'Port', '4');
      |         set_param([gcb '/f32RampOut_preset'], 'Port', '5');
      | 
      |         set_param([gcb '/pIDQReq'], 'Port', '1');
      |         set_param([gcb '/u16LimitFlagQ'], 'Port', '2');
      | 
      |         set_param(gcb,'MaskEnables',{'on','on','off','on','on','on','on','on','on','on','on','on'});
      | 
      |         if (posblk(4) - posblk(2)) > 150
      |           height = 150;
      |           set_param(gcb,'Position',[posblk(1), posblk(2), posblk(3), posblk(2)+height])
      |         end
      |     end
      | else
      |     % shown state variables
      |     if strcmp(get_param([gcb '/u16NSamplesW'], 'BlockType'), 'Ground')
      |         posblk = get_param(gcb, 'Position');
      | 
      |         pos = get_param(    [gcb, '/u16NSamplesW'], 'Position');
      |         orient = get_param( [gcb, '/u16NSamplesW'], 'Orientation');
      |         delete_block(       [gcb, '/u16NSamplesW']);
      |         add_block('built-in/Inport', [gcb, '/u16NSamplesW'], 'Position', pos, 'Orientation', orient, 'OutDataTypeStr', 'uint16');
      | 
      |         pos = get_param(    [gcb, '/f16PropGainQ'], 'Position');
      |         orient = get_param( [gcb, '/f16PropGainQ'], 'Orientation');
      |         delete_block(       [gcb, '/f16PropGainQ']);
      |         add_block('built-in/Inport', [gcb, '/f16PropGainQ'], 'Position', pos, 'Orientation', orient, 'OutDataTypeStr', 'int16');
      | 
      |         pos = get_param(    [gcb, '/f16IntegGainQ'], 'Position');
      |         orient = get_param( [gcb, '/f16IntegGainQ'], 'Orientation');
      |         delete_block(       [gcb, '/f16IntegGainQ']);
      |         add_block('built-in/Inport', [gcb, '/f16IntegGainQ'], 'Position', pos, 'Orientation', orient, 'OutDataTypeStr', 'int16');
      | 
      |         pos = get_param(    [gcb, '/s16PropGainShiftQ'], 'Position');
      |         orient = get_param( [gcb, '/s16PropGainShiftQ'], 'Orientation');
      |         delete_block(       [gcb, '/s16PropGainShiftQ']);
      |         add_block('built-in/Inport', [gcb, '/s16PropGainShiftQ'], 'Position', pos, 'Orientation', orient, 'OutDataTypeStr', 'int16');
      | 
      |         pos = get_param(    [gcb, '/s16IntegGainShiftQ'], 'Position');
      |         orient = get_param( [gcb, '/s16IntegGainShiftQ'], 'Orientation');
      |         delete_block(       [gcb, '/s16IntegGainShiftQ']);
